simulink model "commander_old"  (R2024b)
(part 3 of 3)

    |     set_health_flags(SUBSYSTEM_TYPE_DIFFPRESSURE, present, ~optional_aspd, success, vehicle_status_out_);
    |     ret = success;
    |     return
    | end
    | 
    | %% Check if airspeed is declared valid or not by airspeed selector.
    | if ~isfinite(airspeed_validated.calibrated_airspeed_m_s) && report_fail
    |     sprintf("mavlink_log_critical, Preflight Fail: Airspeed invalid.");
    | end
    | present = true;
    | success = false;
    | set_health_flags(SUBSYSTEM_TYPE_DIFFPRESSURE, present, ~optional_aspd, success, vehicle_status_out_);
    | ret = success;
    | return
    | 
    | %% Check if airspeed is higher than maximally accepted while the vehicle is landed / not flying
    | %% Negative and positive offsets are considered. Do not check anymore while arming because pitot cover
    | %% might have been removed.
    | if max_aspd_check_en && fabsf(airspeed_validated.calibrated_airspeed_m_s) > arming_max_aspd_allowed && ...
    |         prearm && report_fail
    |     sprintf("mavlink_log_critical, Preflight Fail: check Airspeed Cal or pitot");
    | end
    | 
    | present = true;
    | success = false;
    | set_health_flags(SUBSYSTEM_TYPE_DIFFPRESSURE, present, ~optional_aspd, success, vehicle_status_out_);
    | ret = success;
    | return
    | 
    | end
  function ret = rcCheck(is_report_rc_fail, isVTOL):
    | function ret = rcCheck(is_report_rc_fail, isVTOL)
    | 
    | map_fail_count = 0;
    | total_fail_count = 0;
    | 
    | % if VTOL, check transition switch mapping
    | if isVTOL
    |     if RC_MAP_TRANS_SW == 0xffff && is_report_rc_fail
    |         sprintf("mavlink_log_critical, RC_MAP_TRANS_SW PARAMETER MISSING.");
    |         map_fail_count = map_fail_count + 1;
    |     elseif RC_MAP_TRANS_SW < 1
    |         if is_report_rc_fail
    |             sprintf("mavlink_log_critical, Transition switch RC_MAP_TRANS_SW not set.");
    |         end
    |         map_fail_count = map_fail_count + 1;
    |     end
    | 
    |     % first check channel mappings
    |     % 暂不实现
    | 
    |     channels_failed = 0;
    |     count = 0;
    | 
    |     % min values
    |     RC_INPUT_MIN_SETS = [RC1_MIN, RC2_MIN, RC3_MIN, RC4_MIN, RC5_MIN, RC6_MIN, ...
    |         RC7_MIN, RC8_MIN, RC9_MIN, RC10_MIN, RC11_MIN, RC12_MIN, ...
    |         RC13_MIN, RC14_MIN, RC15_MIN, RC16_MIN, RC17_MIN, RC18_MIN];
    | 
    |     % trim values
    |     RC_INPUT_TRIM_SETS = [RC1_TRIM, RC2_TRIM, RC3_TRIM, RC4_TRIM, RC5_TRIM, RC6_TRIM, ...
    |         RC7_TRIM, RC8_TRIM, RC9_TRIM, RC10_TRIM, RC11_TRIM, RC12_TRIM, ...
    |         RC13_TRIM, RC14_TRIM, RC15_TRIM, RC16_TRIM, RC17_TRIM, RC18_TRIM];
    | 
    |     % max values
    |     RC_INPUT_MAX_SETS = [RC1_MAX, RC2_MAX, RC3_MAX, RC4_MAX, RC5_MAX, RC6_MAX, ...
    |         RC7_MAX, RC8_MAX, RC9_MAX, RC10_MAX, RC11_MAX, RC12_MAX, ...
    |         RC13_MAX, RC14_MAX, RC15_MAX, RC16_MAX, RC17_MAX, RC18_MAX];
    | 
    |     % channel reverse
    |     RC_INPUT_REVERSE_SETS = [RC1_REV, RC2_REV, RC3_REV, RC4_REV, RC5_REV, RC6_REV, ...
    |         RC7_REV, RC8_REV, RC9_REV, RC10_REV, RC11_REV, RC12_REV, ...
    |         RC13_REV, RC14_REV, RC15_REV, RC16_REV, RC17_REV, RC18_REV];
    | 
    |     % channel deadzone
    |     RC_INPUT_DEADZONE_SETS = [RC1_DZ, RC2_DZ, RC3_DZ, RC4_DZ, RC5_DZ, RC6_DZ, ...
    |         RC7_DZ, RC8_DZ, RC9_DZ, RC10_DZ, RC11_DZ, RC12_DZ, ...
    |         RC13_DZ, RC14_DZ, RC15_DZ, RC16_DZ, RC17_DZ, RC18_DZ];
    | 
    |     for i = 1:uint8(PX4_INPUT_RC.RC_INPUT_MAX_CHANNELS)
    |         %% 检查MIN值的合理性
    |         if RC_INPUT_MIN_SETS(i) < RC_INPUT_LOWEST_MIN_US
    |             count = count + 1;
    |             if is_report_rc_fail
    |                 sprintf("mavlink_log_critical, RC_ERROR: RC%u_MIN < %d", i, RC_INPUT_LOWEST_MIN_US);
    |             end
    |         end
    | 
    |         %% 检查MAX值的合理性
    |         if RC_INPUT_MAX_SETS(i) > RC_INPUT_HIGHEST_MAX_US
    |             count = count + 1;
    |             if is_report_rc_fail
    |                 sprintf("mavlink_log_critical, RC_ERROR: RC%u_MAX < %d", i, RC_INPUT_HIGHEST_MAX_US);
    |             end
    |         end
    | 
    |         %% 检查TRIM与MIN数值的合理性
    |         if RC_INPUT_TRIM_SETS(i) < RC_INPUT_MIN_SETS(i)
    |             count = count + 1;
    |             if is_report_rc_fail
    |                 sprintf("mavlink_log_critical, RC ERROR: RC%d_TRIM < MIN (%d/%d).", int8(i), int16(RC_INPUT_TRIM_SETS(i)), int16(RC_INPUT_MIN_SETS(i)));
    |             end
    |         end
    | 
    |         %% 检查TRIM与MAX数值的合理性
    |         if RC_INPUT_TRIM_SETS(i) > RC_INPUT_MAX_SETS(i)
    |             count = count + 1;
    |             if is_report_rc_fail
    |                 sprintf("mavlink_log_critical, RC ERROR: RC%d_TRIM > MAX (%d/%d).", int8(i), int16(RC_INPUT_TRIM_SETS(i)), int16(RC_INPUT_MAX_SETS(i)));
    |             end
    |         end
    | 
    |         %% 检查死区的合理性
    |         if RC_INPUT_DEADZONE_SETS(i) > RC_INPUT_MAX_DEADZONE_US
    |             count = count + 1;
    |             if is_report_rc_fail
    |                 sprintf("mavlink_log_critical, RC ERROR: RC%d_DZ > %d.", int8(i), int16(RC_INPUT_MAX_DEADZONE_US));
    |             end
    |         end
    | 
    |         total_fail_count = total_fail_count + count;
    | 
    |     end
    | 
    | end
    | 
    | ret = total_fail_count;
    | 
    | end % function end
  function ret = powerCheck(report_power_fail, prearm):
    | function ret = powerCheck(report_power_fail, prearm)
    | 
    | ret = true;
    | 
    | if ~prearm
    |     % Ignore power check after arming.
    |     ret = true;
    |     return
    | end
    | 
    | if vehicle_status_out_.hil_state == PX4_VEHICLE_STATUS.HIL_STATE_ON
    |     % Ignore power check in HITL.
    |     ret = true;
    |     return
    | end
    | 
    | if system_power.timestamp ~= 0
    |     %% system_power主题有效
    |     required_power_module_count = 0;
    |     required_power_module_count = COM_POWER_COUNT;
    | 
    |     % Check avionics rail voltages (if USB isn't connected)
    |     if ~system_power.usb_connected
    | 
    |         avionics_power_rail_voltage = system_power.voltage5v_v;
    | 
    |         if avionics_power_rail_voltage < 4.5
    |             ret = false;
    |             if report_power_fail
    |                 sprintf("mavlink_log_critical, Preflight Fail: Avionics Power low: %6.2f Volt", single(avionics_power_rail_voltage));
    |             end
    |         elseif avionics_power_rail_voltage < 4.8 && report_power_fail
    |             sprintf("mavlink_log_critical, CAUTION: Avionics Power low: %6.2f Volt", single(avionics_power_rail_voltage));
    |         elseif avionics_power_rail_voltage > 5.4 && report_power_fail
    |             sprintf("mavlink_log_critical, CAUTION: Avionics Power high: %6.2f Volt", single(avionics_power_rail_voltage));
    |         end
    | 
    |         power_module_count = countSetBits(system_power.brick_valid);
    | 
    |         if power_module_count < required_power_module_count
    |             ret = false;
    |             if report_power_fail
    |                 sprintf("mavlink_log_critical, Power redundancy not met: %d instead of %d PRId32", int8(power_module_count), int8(required_power_module_count));
    |             end
    |         end
    | 
    |     elseif report_power_fail
    |         %% 主题无效
    |         sprintf("mavlink_log_critical, system power unavailable");
    |         ret = false;
    |         return
    | 
    |     end
    | 
    | end
    | 
    | end
    | 
    | %% 统计uint8的数据n中有多少位置1
    | function ret = countSetBits(n)
    | 
    | count = 0;
    | 
    | while n
    |     if bitand(uint8(n), uint8(1)) == 1
    |         count = count + 1;
    |     end
    |     n = bitshift(n, -1);
    | end
    | 
    | ret = count;
    | 
    | end
  function ret = failureDetectorCheck(report_failure_fail):
    | function ret = failureDetectorCheck(report_failure_fail)
    | 
    | ret = true;
    | 
    | % Ignore failure detector check after arming
    | if ~prearm_
    |     ret = true;
    |     return
    | end
    | 
    | if vehicle_status_out_.failure_detector_status ~= PX4_VEHICLE_STATUS.FAILURE_NONE
    | 
    |     if report_failure_fail
    |         if bitand(vehicle_status_out_.failure_detector_status, uint8(PX4_VEHICLE_STATUS.FAILURE_ROLL))
    |             sprintf("mavlink_log_critical, Preflight Fail: Roll failure detected");
    |         end
    | 
    |         if bitand(vehicle_status_out_.failure_detector_status, uint8(PX4_VEHICLE_STATUS.FAILURE_PITCH))
    |             sprintf("mavlink_log_critical, Preflight Fail: Pitch failure detected");
    |         end
    | 
    |         if bitand(vehicle_status_out_.failure_detector_status, uint8(PX4_VEHICLE_STATUS.FAILURE_ALT))
    |             sprintf("mavlink_log_critical, Preflight Fail: Altitude failure detected");
    |         end
    | 
    |         if bitand(vehicle_status_out_.failure_detector_status, uint8(PX4_VEHICLE_STATUS.FAILURE_EXT))
    |             sprintf("mavlink_log_critical, Preflight Fail: Parachute failure detected");
    |         end
    | 
    |         if bitand(vehicle_status_out_.failure_detector_status, uint8(PX4_VEHICLE_STATUS.FAILURE_ARM_ESC))
    |             sprintf("mavlink_log_critical, Preflight Fail: ESC failure detected");
    |         end
    |     end
    | 
    |     ret = false;
    |     return
    | 
    | end
    | 
    | ret = true;
    | return
    | 
    | end
  function ret = ekf2Check(report_ekf_fail):
    | function ret = ekf2Check(report_ekf_fail)
    | 
    | ret = true; % start with a pass and change to a fail if any test fails
    | 
    | mag_strength_check_enabled  = COM_ARM_MAG_STR;
    | hgt_test_ratio_limit        = COM_ARM_EKF_HGT;
    | vel_test_ratio_limit        = COM_ARM_EKF_VEL;
    | pos_test_ratio_limit        = COM_ARM_EKF_POS;
    | mag_test_ratio_limit        = COM_ARM_EKF_YAW;
    | arm_without_gps             = COM_ARM_WO_GPS;
    | 
    | gps_success = true;
    | gps_present = true;
    | 
    | % Get estimator status data if available and exit with a fail recorded if not
    | if vehicle_status_out_.timestamp == 0
    |     ret = false;
    |     set_health_flags(SUBSYSTEM_TYPE_GPS, gps_present, ~arm_without_gps, ret, vehicle_status_out_);
    |     return
    | end
    | 
    | % Check if preflight check performed by estimator has failed
    | if estimator_status.pre_flt_fail_innov_heading || estimator_status.pre_flt_fail_innov_vel_horiz || ...
    |         estimator_status.pre_flt_fail_innov_vel_vert || estimator_status.pre_flt_fail_innov_height
    | 
    |     if report_ekf_fail
    |         if estimator_status.pre_flt_fail_innov_heading
    |             sprintf("mavlink_log_critical, Preflight Fail: heading estimate not stable");
    |         elseif estimator_status.pre_flt_fail_innov_vel_horiz
    |             sprintf("mavlink_log_critical, Preflight Fail: horizontal velocity estimate not stable");
    |         elseif estimator_status.pre_flt_fail_innov_vel_vert
    |             sprintf("mavlink_log_critical, Preflight Fail: vertical velocity estimate not stable");
    |         elseif estimator_status.pre_flt_fail_innov_height
    |             sprintf("mavlink_log_critical, Preflight Fail: height estimate not stable");
    |         end
    |     end
    | 
    |     ret = false;
    |     set_health_flags(SUBSYSTEM_TYPE_GPS, gps_present, ~arm_without_gps, ret, vehicle_status_out_);
    |     return
    | 
    | end
    | 
    | %% 磁力计干扰检查
    | if mag_strength_check_enabled == 1 && estimator_status.pre_flt_fail_mag_field_disturbed
    |     if report_ekf_fail
    |         sprintf("mavlink_log_critical, Preflight Fail: strong magnetic interference detected");
    |     end
    |     ret = false;
    |     set_health_flags(SUBSYSTEM_TYPE_GPS, gps_present, ~arm_without_gps, ret, vehicle_status_out_);
    |     return
    | end
    | 
    | %% check vertical position innovation test ratio
    | if estimator_status.hgt_test_ratio > hgt_test_ratio_limit
    |     if report_ekf_fail
    |         sprintf("Preflight Fail: Height estimate error");
    |     end
    |     ret = false;
    |     set_health_flags(SUBSYSTEM_TYPE_GPS, gps_present, ~arm_without_gps, ret, vehicle_status_out_);
    |     return
    | end
    | 
    | %% check velocity innovation test ratio
    | if estimator_status.vel_test_ratio > vel_test_ratio_limit
    |     if report_ekf_fail
    |         sprintf("mavlink_log_critical, Preflight Fail: Velocity estimate error");
    |         ret = false;
    |         set_health_flags(SUBSYSTEM_TYPE_GPS, gps_present, ~arm_without_gps, ret, vehicle_status_out_);
    |         return
    |     end
    | end
    | 
    | %% check horizontal position innovation test ratio
    | if estimator_status.pos_test_ratio > pos_test_ratio_limit
    |     if report_ekf_fail
    |         sprintf("Preflight Fail: Position estimate error");
    |     end
    |     ret = false;
    |     set_health_flags(SUBSYSTEM_TYPE_GPS, gps_present, ~arm_without_gps, ret, vehicle_status_out_);
    |     return
    | end
    | 
    | %% check magnetometer innovation test ratio
    | if estimator_status.mag_test_ratio > mag_test_ratio_limit
    |     if report_ekf_fail
    |         sprintf("Preflight Fail: Yaw estimate error");
    |     end
    |     ret = false;
    |     set_health_flags(SUBSYSTEM_TYPE_GPS, gps_present, ~arm_without_gps, ret, vehicle_status_out_);
    |     return
    | end
    | 
    | %% If GPS aiding is required, declare fault condition if the required GPS quality checks are failing
    | ekf_gps_fusion = bitand(estimator_status.control_mode_flags, bitshift(1, PX4_ESTIMATOR_STATUS.CS_GPS));
    | ekf_gps_check_fail = estimator_status.gps_check_fail_flags > 0;
    | 
    | gps_success = ekf_gps_fusion; % default to success if gps data is fused
    | 
    | if ekf_gps_check_fail
    | 
    |     if report_ekf_fail
    |         % Only report the first failure to avoid spamming
    |         if bitand(estimator_status.gps_check_fail_flags, bitshift(1, PX4_ESTIMATOR_STATUS.GPS_CHECK_FAIL_GPS_FIX)) && ~arm_without_gps
    |             sprintf("mavlink_log_critical, Preflight Fail: GPS fix too low");
    |         elseif bitand(estimator_status.gps_check_fail_flags, bitshift(1, PX4_ESTIMATOR_STATUS.GPS_CHECK_FAIL_MIN_SAT_COUNT)) && ~arm_without_gps
    |             sprintf("mavlink_log_critical, Preflight Fail: not enough GPS Satellites");
    |         elseif bitand(estimator_status.gps_check_fail_flags, bitshift(1, PX4_ESTIMATOR_STATUS.GPS_CHECK_FAIL_MAX_PDOP)) && ~arm_without_gps
    |             sprintf("mavlink_log_critical, Preflight Fail: GPS PDOP too high");
    |         elseif bitand(estimator_status.gps_check_fail_flags, bitshift(1, PX4_ESTIMATOR_STATUS.GPS_CHECK_FAIL_MAX_HORZ_ERR)) && ~arm_without_gps
    |             sprintf("mavlink_log_critical, Preflight Fail: GPS Horizontal Pos Error too high");
    |         elseif bitand(estimator_status.gps_check_fail_flags, bitshift(1, PX4_ESTIMATOR_STATUS.GPS_CHECK_FAIL_MAX_VERT_ERR)) && ~arm_without_gps
    |             sprintf("mavlink_log_critical, Preflight Fail: GPS Vertical Pos Error too high");
    |         elseif bitand(estimator_status.gps_check_fail_flags, bitshift(1, PX4_ESTIMATOR_STATUS.GPS_CHECK_FAIL_MAX_SPD_ERR)) && ~arm_without_gps
    |             sprintf("mavlink_log_critical, Preflight Fail: GPS Speed Accuracy too low");
    |         elseif bitand(estimator_status.gps_check_fail_flags, bitshift(1, PX4_ESTIMATOR_STATUS.GPS_CHECK_FAIL_MAX_HORZ_DRIFT)) && ~arm_without_gps
    |             sprintf("mavlink_log_critical, Preflight Fail: GPS Horizontal Pos Drift too high");
    |         elseif bitand(estimator_status.gps_check_fail_flags, bitshift(1, PX4_ESTIMATOR_STATUS.GPS_CHECK_FAIL_MAX_VERT_DRIFT)) && ~arm_without_gps
    |             sprintf("mavlink_log_critical, Preflight Fail: GPS Vertical Pos Drift too high");
    |         elseif bitand(estimator_status.gps_check_fail_flags, bitshift(1, PX4_ESTIMATOR_STATUS.GPS_CHECK_FAIL_MAX_HORZ_SPD_ERR)) && ~arm_without_gps
    |             sprintf("mavlink_log_critical, Preflight Fail: GPS Hor Speed Drift too high");
    |         elseif bitand(estimator_status.gps_check_fail_flags, bitshift(1, PX4_ESTIMATOR_STATUS.GPS_CHECK_FAIL_MAX_VERT_SPD_ERR)) && ~arm_without_gps
    |             sprintf("mavlink_log_critical, Preflight Fail: GPS Vert Speed Drift too high");
    |         else
    |             if ~ekf_gps_fusion
    |                 % Likely cause unknown
    |                 sprintf("mavlink_log_critical, Preflight Fail: Estimator not using GPS");
    |                 gps_present = false;
    |             else
    |                 % if we land here there was a new flag added and the code not updated. Show a generic message.
    |                 sprintf("mavlink_log_critical, Preflight Fail: Poor GPS Quality");
    |             end
    |         end
    | 
    |         gps_success = false;
    | 
    |         if ~arm_without_gps
    |             ret = false;
    |             set_health_flags(SUBSYSTEM_TYPE_GPS, gps_present, ~arm_without_gps, gps_success, vehicle_status_out_);
    |             return
    |         end
    |     end
    | 
    | end
    | 
    | end % function end
  function ret = ekf2CheckSensorBias(report_bias_fail):
    | function ret = ekf2CheckSensorBias(report_bias_fail)
    | 
    | % Get estimator states data if available and exit with a fail recorded if not
    | % uORB::SubscriptionData<estimator_selector_status_s> estimator_selector_status_sub{ORB_ID(estimator_selector_status)};
    | % uORB::SubscriptionData<estimator_sensor_bias_s> estimator_sensor_bias_sub{ORB_ID(estimator_sensor_bias), estimator_selector_status_sub.get().primary_instanceend};
    | 
    | if (getSimulationTime*1e+6 - estimator_sensor_bias.timestamp) < 30*1e+6
    | 
    |     %% check accelerometer bias estimates
    |     if estimator_sensor_bias.accel_bias_valid
    |         ekf_ab_test_limit = 0.75 * estimator_sensor_bias.accel_bias_limit;
    |         for axis_index = 1:3
    |             % allow for higher uncertainty in estimates for axes that are less observable to prevent false positives
    |             % adjust test threshold by 3-sigma
    |             test_uncertainty = 3.0 * sqrt(max(estimator_sensor_bias.accel_bias_variance(axis_index), 0.0));
    |             if abs(estimator_sensor_bias.accel_bias(axis_index)) > (ekf_ab_test_limit + test_uncertainty)
    |                 if report_bias_fail
    |                     sprintf("PX4_ERR, accel bias (axis %d): |%f| > %f + %f", int8(axis_index), ...
    |                         single(estimator_sensor_bias.accel_bias(axis_index)), single(ekf_ab_test_limit), single(test_uncertainty));
    |                     sprintf("mavlink_log_critical, Preflight Fail: High Accelerometer Bias");
    |                 end
    |                 ret = false;
    |                 return
    |             end
    |         end
    |     end
    | 
    |     %% check gyro bias estimates
    |     if estimator_sensor_bias.gyro_bias_valid
    |         ekf_gb_test_limit = 0.75 * estimator_sensor_bias.gyro_bias_limit;
    |         for axis_index = 1:3
    |             % allow for higher uncertainty in estimates for axes that are less observable to prevent false positives
    |             % adjust test threshold by 3-sigma
    |             test_uncertainty = 3.0 * sqrt(max(estimator_sensor_bias.gyro_bias_variance(axis_index), 0.0));
    |             if abs(estimator_sensor_bias.gyro_bias(axis_index)) > (ekf_gb_test_limit + test_uncertainty)
    |                 if report_bias_fail
    |                     sprintf("PX4_ERR, gyro bias (axis %d): |%f| > %f + %f", int8(axis_index), ...
    |                         single(estimator_sensor_bias.gyro_bias(axis_index)), single(ekf_gb_test_limit), single(test_uncertainty));
    |                     sprintf("mavlink_log_critical, Preflight Fail: High Gyro Bias");
    |                 end
    |                 ret = false;
    |                 return
    |             end
    |         end
    |     end
    | 
    | end
    | 
    | ret = true;
    | 
    | end % function end
  function ret = manualCheck(report_manual_fail):
    | function ret = manualCheck(report_manual_fail)
    | 
    | ret = true;
    | 
    | if manual_control_switches.timestamp ~= 0
    | 
    |     % check action switches
    |     if manual_control_switches.return_switch == PX4_MANUAL_CONTROL_SWITCHES.SWITCH_POS_ON
    |         ret = false;
    |         if report_manual_fail
    |             sprintf("mavlink_log_critical, Failure: RTL switch engaged");
    |         end
    |     end
    | 
    |     if manual_control_switches.kill_switch == PX4_MANUAL_CONTROL_SWITCHES.SWITCH_POS_ON
    |         ret = false;
    |         if report_manual_fail
    |             sprintf("mavlink_log_critical, Failure: Kill switch engaged");
    |         end
    |     end
    | 
    |     if manual_control_switches.gear_switch == PX4_MANUAL_CONTROL_SWITCHES.SWITCH_POS_ON
    |         ret = false;
    |         if (report_manual_fail)
    |             sprintf("mavlink_log_critical, Failure: Landing gear switch set in UP position");
    |         end
    |     end
    |     
    | end
    | 
    | end
  function ret = cpuCheck(report_cpu_fail):
    | function ret = cpuCheck(report_cpu_fail)
    | 
    | ret = true;
    | 
    | cpuload_percent_max = COM_CPU_MAX;
    | 
    | if cpuload_percent_max > 0.0
    | 
    |     if (getSimulationTime*1e+6 - cpuload.timestamp) > 2*1e+6
    |         ret = false;
    |         if report_cpu_fail
    |             sprintf("mavlink_log_critical, Fail: No CPU load information");
    |         end
    |     end
    | 
    |     cpuload_percent = cpuload.load * 100;
    | 
    |     if cpuload_percent > cpuload_percent_max
    |         ret = false;
    |         if report_cpu_fail
    |             sprintf("mavlink_log_critical, Fail: CPU load too high: %f", single(cpuload_percent));
    |         end
    |     end
    | 
    | end
    | 
    | end
  function ret = is_fixed_wing(current_status):
    | function ret = is_fixed_wing(current_status)
    | 
    | ret = current_status.system_type == VEHICLE_TYPE_FIXED_WING;
    | 
    | end
  function ret = is_multirotor(current_status):
    | function ret = is_multirotor(current_status)
    | 
    | ret = ((current_status.system_type == VEHICLE_TYPE_QUADROTOR) || ...
    |     (current_status.system_type == VEHICLE_TYPE_HEXAROTOR) || ...
    |     (current_status.system_type == VEHICLE_TYPE_OCTOROTOR) || ...
    |     (current_status.system_type == VEHICLE_TYPE_TRICOPTER));
    | 
    | end
  function ret = is_ground_rover(current_status):
    | function ret = is_ground_rover(current_status)
    | 
    | ret = current_status.system_type == VEHICLE_TYPE_GROUND_ROVER;
    | 
    | end
  function get_circuit_breaker_params:
    | function get_circuit_breaker_params()
    | 
    | vehicle_status_flags_out_.circuit_breaker_engaged_power_check = (CBRK_SUPPLY_CHK == CBRK_SUPPLY_CHK_KEY);
    | vehicle_status_flags_out_.circuit_breaker_engaged_usb_check = (CBRK_USB_CHK == CBRK_USB_CHK_KEY);
    | vehicle_status_flags_out_.circuit_breaker_engaged_airspd_check = (CBRK_AIRSPD_CHK == CBRK_AIRSPD_CHK_KEY);
    | vehicle_status_flags_out_.circuit_breaker_engaged_enginefailure_check = (CBRK_ENGINEFAIL == CBRK_ENGINEFAIL_KEY);
    | vehicle_status_flags_out_.circuit_breaker_flight_termination_disabled = (CBRK_FLIGHTTERM == CBRK_FLIGHTTERM_KEY);
    | vehicle_status_flags_out_.circuit_breaker_engaged_posfailure_check = (CBRK_VELPOSERR == CBRK_VELPOSERR_KEY);
    | vehicle_status_flags_out_.circuit_breaker_vtol_fw_arming_check = (CBRK_VTOLARMING == CBRK_VTOLARMING_KEY);
    | 
    | end
  function update_vtol_status:
    | function update_vtol_status()
    | 
    | % vtol status changed
    | vehicle_status_out_.vtol_fw_permanent_stab = vtol_status.fw_permanent_stab;
    | 
    | % Make sure that this is only adjusted if vehicle really is of type vtol
    | if is_vtol(vehicle_status_out_)
    | 
    |     % Check if there has been any change while updating the flags
    |     if vtol_status.vtol_in_rw_mode % 转换和多旋翼阶段
    |         new_vehicle_type = uint8(PX4_VEHICLE_STATUS.VEHICLE_TYPE_ROTARY_WING);
    |     else  % 纯固定翼
    |         new_vehicle_type = uint8(PX4_VEHICLE_STATUS.VEHICLE_TYPE_FIXED_WING);
    |     end
    | 
    |     if new_vehicle_type ~= vehicle_status_out_.vehicle_type
    |         vehicle_status_out_.vehicle_type = new_vehicle_type;
    |         g_status_changed = true;
    |     end
    | 
    |     if vehicle_status_out_.in_transition_mode ~= vtol_status.vtol_in_trans_mode
    |         vehicle_status_out_.in_transition_mode = vtol_status.vtol_in_trans_mode;
    |         g_status_changed = true;
    |     end
    | 
    |     if vehicle_status_out_.in_transition_to_fw ~= vtol_status.in_transition_to_fw
    |         vehicle_status_out_.in_transition_to_fw = vtol_status.in_transition_to_fw;
    |         g_status_changed = true;
    |     end
    | 
    |     if vehicle_status_flags_out_.vtol_transition_failure ~= vtol_status.vtol_transition_failsafe
    |         vehicle_status_flags_out_.vtol_transition_failure = vtol_status.vtol_transition_failsafe;
    |         g_status_changed = true;
    |     end
    | 
    |     should_soft_stop = (vehicle_status_out_.vehicle_type ~= uint8(PX4_VEHICLE_STATUS.VEHICLE_TYPE_ROTARY_WING));
    | 
    |     if actuator_armed_out_.soft_stop ~= should_soft_stop
    |         actuator_armed_out_.soft_stop = should_soft_stop;
    |         g_status_changed = true;
    |     end
    | 
    | end
    | 
    | end % function end
  function last_esc_updated = esc_status_check:
    | function last_esc_updated = esc_status_check
    | 
    | persistent last_esc_online_flags
    | persistent last_esc_failure
    | 
    | if isempty(last_esc_online_flags)
    |     last_esc_online_flags = uint8(0);
    | end
    | 
    | if isempty(last_esc_failure)
    |     last_esc_failure = uint8(zeros(1, uint8(PX4_ESC_STATUS.CONNECTED_ESC_MAX)));
    | end
    | 
    | last_esc_updated = esc_status.timestamp;
    | 
    | if esc_status.esc_count > 0
    | 
    |     online_bitmask = bitshift(1, esc_status.esc_count) - 1;
    | 
    |     %% Check if ALL the ESCs are online
    |     if online_bitmask == esc_status.esc_online_flags
    |         vehicle_status_flags_out_.condition_escs_error = false;
    |         last_esc_online_flags = esc_status.esc_online_flags;
    |     elseif esc_status.esc_online_flags == last_esc_online_flags
    |         % Avoid checking the status if the flags are the same or if the mixer has not yet been loaded in the ESC driver
    |         vehicle_status_flags_out_.condition_escs_error = true;
    |     elseif esc_status.esc_online_flags < last_esc_online_flags
    |         % Only warn the user when an ESC goes from ONLINE to OFFLINE. This is done to prevent showing Offline ESCs warnings at boot
    |         for index = 1:esc_status.esc_count
    |             if bitand(esc_status.esc_online_flags, bitshift(1,index-1)) == 0
    |                 sprintf("mavlink_log_critical, %d offline", int8(index));
    |             end
    |         end
    |         last_esc_online_flags = esc_status.esc_online_flags;
    |         vehicle_status_flags_out_.condition_escs_error = true;
    |     end
    | 
    |     vehicle_status_flags_out_.condition_escs_failure = false;
    | 
    |     for index = 1:esc_status.esc_count
    | 
    |         if esc_status.esc(index).failures > PX4_ESC_REPORT.FAILURE_NONE
    |             vehicle_status_flags_out_.condition_escs_failure = true;
    | 
    |             if esc_status.esc(index).failures ~= last_esc_failure(index)
    | 
    |                 if bitand(esc_status.esc(index).failures, uint8(PX4_ESC_REPORT.FAILURE_OVER_CURRENT_MASK))
    |                     sprintf("mavlink_log_critical ESC%d: over current", int8(index));
    |                 end
    | 
    |                 if bitand(esc_status.esc(index).failures, uint8(PX4_ESC_REPORT.FAILURE_OVER_VOLTAGE_MASK))
    |                     sprintf("mavlink_log_critical ESC%d: over voltage", int8(index));
    |                 end
    | 
    |                 if bitand(esc_status.esc(index).failures, uint8(PX4_ESC_REPORT.FAILURE_OVER_TEMPERATURE_MASK))
    |                     sprintf("mavlink_log_critical ESC%d: over temperature", int8(index));
    |                 end
    | 
    |                 if bitand(esc_status.esc(index).failures, uint8(PX4_ESC_REPORT.FAILURE_OVER_RPM_MASK))
    |                     sprintf("mavlink_log_critical ESC%d: over RPM", int8(index));
    |                 end
    | 
    |                 if bitand(esc_status.esc(index).failures, uint8(PX4_ESC_REPORT.FAILURE_INCONSISTENT_CMD_MASK))
    |                     sprintf("mavlink_log_critical ESC%d: command inconsistency", int8(index));
    |                 end
    | 
    |                 if bitand(esc_status.esc(index).failures, uint8(PX4_ESC_REPORT.FAILURE_MOTOR_STUCK_MASK))
    |                     sprintf("mavlink_log_critical ESC%d: motor stuck", int8(index));
    |                 end
    | 
    |                 if bitand(esc_status.esc(index).failures, uint8(PX4_ESC_REPORT.FAILURE_GENERIC_MASK))
    |                     sprintf("mavlink_log_critical ESC%d: generic failure - code %d", int8(index), int16(esc_status.esc(index).esc_state));
    |                 end
    | 
    |             end
    | 
    |             last_esc_failure(index) = esc_status.esc(index).failures;
    |         end
    | 
    |     end
    | 
    | end
    | 
    | end % function end
  function ekf_status_check:
    | function ekf_status_check()
    | 
    | % persistent parameters
    | persistent heading_reset_counter
    | persistent time_last_innov_fail
    | persistent time_last_innov_pass
    | 
    | if isempty(heading_reset_counter)
    |     heading_reset_counter = uint8(0);
    | end
    | 
    | if isempty(time_last_innov_fail)
    |     time_last_innov_fail = uint64(0);
    | end
    | 
    | if isempty(time_last_innov_pass)
    |     time_last_innov_pass = uint64(0);
    | end
    | 
    | % Check if quality checking of position accuracy and consistency is to be performed
    | % circuit_breaker_engaged_posfailure_check: set to true when the position valid checks have been disabled
    | run_quality_checks = ~vehicle_status_flags_out_.circuit_breaker_engaged_posfailure_check;
    | if local_position.heading_reset_counter ~= heading_reset_counter
    |     if vehicle_status_flags_out_.condition_home_position_valid
    |         updateHomePositionYaw(home_position.yaw + local_position.delta_heading);
    |     end
    |     heading_reset_counter = local_position.heading_reset_counter;
    | end
    | 
    | mag_fault_prev = bitand(estimator_status.control_mode_flags, bitshift(1, PX4_ESTIMATOR_STATUS.CS_MAG_FAULT));
    | 
    | %% use primary estimator_status, but we use only one ekf
    | if hasChanged(estimator_status.timestamp)
    | 
    |     % Check for a magnetomer fault and notify the user
    |     mag_fault = bitand(estimator_status.control_mode_flags, bitshift(1, PX4_ESTIMATOR_STATUS.CS_MAG_FAULT));
    |     if ~mag_fault_prev && mag_fault
    |         sprintf("mavlink_log_critical, Stopping compass use~ Check calibration on landing");
    |         set_health_flags(SUBSYSTEM_TYPE_MAG, true, true, false, vehicle_status_out_);
    |     end
    | 
    |     % Check estimator status for signs of bad yaw induced post takeoff navigation failure
    |     % for a short time interval after takeoff.
    |     % Most of the time, the drone can recover from a bad initial yaw using GPS-inertial
    |     % heading estimation (yaw emergency estimator) or GPS heading (fixed wings only), but
    |     % if this does not fix the issue we need to stop using a position controlled
    |     % mode to prevent flyaway crashes.
    |     if run_quality_checks && (vehicle_status_out_.vehicle_type == PX4_VEHICLE_STATUS.VEHICLE_TYPE_ROTARY_WING)
    | 
    |         if vehicle_status_out_.arming_state == PX4_VEHICLE_STATUS.ARMING_STATE_STANDBY
    |             nav_test_failed_ = false;
    |             nav_test_passed_ = false;
    |         else
    |             if ~nav_test_passed_
    |                 % Both test ratios need to pass/fail together to change the nav test status
    |                 innovation_pass = (estimator_status.vel_test_ratio < 1.0) && (estimator_status.pos_test_ratio < 1.0) && ...
    |                     (estimator_status.vel_test_ratio > eps) && (estimator_status.pos_test_ratio > eps);
    |                 innovation_fail = (estimator_status.vel_test_ratio >= 1.0) && (estimator_status.pos_test_ratio >= 1.0);
    | 
    |                 if innovation_pass
    |                     %% innovation_pass
    |                     time_last_innov_pass = uint64(getSimulationTime*1e+6);
    |                     % if nav status is unconfirmed, confirm yaw angle as passed after 30 seconds or achieving 5 m/s of speed
    |                     sufficient_time = (vehicle_status_out_.takeoff_time ~= 0) && ...
    |                         (uint64(getSimulationTime*1e+6 - vehicle_status_out_.takeoff_time) > 30*1e+6);
    |                     sufficient_speed = norm([local_position.vx, local_position.vy]) > 5.0;
    |                     % Even if the test already failed, allow it to pass if it did not fail during the last 10 seconds
    |                     if (uint64(getSimulationTime*1e+6 - time_last_innov_fail) > 10*1e+6) && ...
    |                             (sufficient_time || sufficient_speed)
    |                         nav_test_passed_ = true;
    |                         nav_test_failed_ = false;
    |                     end
    | 
    |                 elseif innovation_fail
    |                     %% innovation_fail
    |                     time_last_innov_fail = uint64(getSimulationTime*1e+6);
    |                     if (~nav_test_failed_ && uint64(getSimulationTime*1e+6) - time_last_innov_pass) > 2*1e+6
    |                         % if the innovation test has failed continuously, declare the nav as failed
    |                         nav_test_failed_ = true;
    |                         sprintf("mavlink_log_emergency, Navigation failure~ Land and recalibrate sensors");
    |                     end
    |                 end
    |             end
    |         end
    |     end
    | 
    | end
    | 
    | %% run position and velocity accuracy checks
    | % Check if quality checking of position accuracy and consistency is to be performed
    | if run_quality_checks
    |     UpdateEstimateValidity();
    | end
    | vehicle_status_flags_out_.condition_local_altitude_valid = local_position.z_valid && ...
    |     (uint64(getSimulationTime*1e+6) - local_position.timestamp) < (COM_POS_FS_DELAY*1e+6);
    | 
    | %% attitude
    | q = vehicle_attitude.q;
    | q_norm = q/norm(q);
    | vehicle_status_flags_out_.condition_attitude_valid = (uint64(getSimulationTime*1e+6) - vehicle_attitude.timestamp) < 1e+6 && ...
    |     norm(q-q_norm) < eps;
    | 
    | %% angular velocity
    | vehicle_status_flags_out_.condition_angular_velocity_valid = ...
    |     (uint64(getSimulationTime*1e+6) - angular_velocity.timestamp) < 1e+6 && ...
    |     isfinite(angular_velocity.xyz(1)) && ...
    |     isfinite(angular_velocity.xyz(2)) && ...
    |     isfinite(angular_velocity.xyz(3));
    | 
    | end % function end
    | 
    | %% updateHomePositionYaw
    | function updateHomePositionYaw(yaw)
    | 
    | home_position_out_.yaw = yaw;
    | home_position_out_.timestamp = uint64(getSimulationTime*1e+6);
    | 
    | end
    | 
    | %% UpdateEstimateValidity
    | function UpdateEstimateValidity()
    | 
    | % COM_POS_FS_EPH: This is the horizontal position error (EPH) threshold that will trigger a failsafe.
    | % The default is appropriate for a multicopter. Can be increased for a fixed-wing.
    | % Default: 5m
    | lpos_eph_threshold_adj = COM_POS_FS_EPH;
    | 
    | % relax local position eph threshold in operator controlled position mode
    | if (internal_state_out_.main_state == PX4_COMMANDER_STATE.MAIN_STATE_POSCTL) && ...
    |         ((vehicle_status_out_.nav_state == PX4_VEHICLE_STATUS.NAVIGATION_STATE_ALTCTL) || ...
    |         (vehicle_status_out_.nav_state == PX4_VEHICLE_STATUS.NAVIGATION_STATE_POSCTL))
    | 
    |     % Set the allowable position uncertainty based on combination of flight and estimator state
    |     % When we are in a operator demanded position control mode and are solely reliant on optical flow,
    |     % do not check position error because it will gradually increase throughout flight and the operator will compensate for the drift
    |     reliant_on_opt_flow = (bitand(estimator_status.control_mode_flags, bitshift(1, PX4_ESTIMATOR_STATUS.CS_OPT_FLOW)) && ...
    |         ~bitand(estimator_status.control_mode_flags, bitshift(1, PX4_ESTIMATOR_STATUS.CS_GPS)) && ...
    |         ~bitand(estimator_status.control_mode_flags, bitshift(1, PX4_ESTIMATOR_STATUS.CS_EV_POS)));
    | 
    |     if reliant_on_opt_flow
    |         lpos_eph_threshold_adj = single(inf);
    |     end
    | end
    | 
    | vehicle_status_flags_out_.condition_global_position_valid = ...
    |     check_posvel_validity(local_position.xy_valid && ~nav_test_failed_, ...
    |     global_position.eph, COM_POS_FS_EPH, ...
    |     global_position.timestamp, ...
    |     last_gpos_fail_time_us_, gpos_probation_time_us_, ...
    |     vehicle_status_flags_out_.condition_global_position_valid);
    | 
    | vehicle_status_flags_out_.condition_local_position_valid = ...
    |     check_posvel_validity(local_position.xy_valid && ~nav_test_failed_, ...
    |     local_position.eph, lpos_eph_threshold_adj, local_position.timestamp, ...
    |     last_lpos_fail_time_us_, lpos_probation_time_us_, ...
    |     vehicle_status_flags_out_.condition_local_position_valid);
    | 
    | vehicle_status_flags_out_.condition_local_velocity_valid = ...
    |     check_posvel_validity(local_position.v_xy_valid && ~nav_test_failed_, ...
    |     local_position.evh, COM_VEL_FS_EVH, local_position.timestamp, ...
    |     last_lvel_fail_time_us_, lvel_probation_time_us_, ...
    |     vehicle_status_flags_out_.condition_local_velocity_valid);
    | 
    | end
  function [batt_warn, batt_warn_inc_while_armed] = battery_check:
    | function [batt_warn, batt_warn_inc_while_armed] = battery_check()
    | 
    | batt_warn = uint8(0);
    | batt_warn_inc_while_armed = false;
    | 
    | if hasChanged(battery_status.timestamp)
    |     
    |     % 此处假定有1块电池connected
    |     num_connected_batteries = 1;
    |     
    |     % 假定所有的电池全为一样的，batteries此处设置为1块电池
    |     for i = 1:num_connected_batteries
    |         batteries(i) = battery_status;
    |     end
    |     
    |     worst_warning = uint8(PX4_BATTERY_STATUS.BATTERY_WARNING_NONE);
    |     oldest_update = uint64(getSimulationTime * 1e+6);
    |     
    |     battery_current_ = single(0.0);
    |     battery_level = single(0.0);
    |     
    |     % Only iterate over connected batteries. We don't care if a disconnected battery is not regularly publishing.
    |     for i = 1:num_connected_batteries
    |         if (batteries(i).warning > worst_warning)
    |             worst_warning = batteries(i).warning;
    |         end
    |         
    |         current_time_us = uint64(getSimulationTime * 1e+6);
    |         if (current_time_us - batteries(i).timestamp) > (current_time_us - oldest_update)
    |             oldest_update = batteries(i).timestamp;
    |         end
    |         
    |         % Sum up current from all batteries.
    |         battery_current_ = battery_current_ + batteries(i).current_filtered_a;
    |         
    |         % average levels from all batteries
    |         battery_level = battery_level + batteries(i).remaining;
    |     end
    |     
    |     battery_level = battery_level / num_connected_batteries;
    |     battery_usage_to_home = single(0.0);
    |     
    |     if uint64(getSimulationTime*1e+6) - rtl_flight_time.timestamp < 2*1e+6
    |         battery_usage_to_home = rtl_flight_time.rtl_limit_fraction;
    |     end
    |     
    |     battery_range_warning = uint8(PX4_BATTERY_STATUS.BATTERY_WARNING_NONE);
    | 
    |     if isfinite(battery_usage_to_home)
    |         
    |         battery_at_home = battery_level - battery_usage_to_home;
    |         if battery_at_home < BAT_CRIT_THR
    |             battery_range_warning = uint8(PX4_BATTERY_STATUS.BATTERY_WARNING_CRITICAL);
    |         elseif battery_at_home < BAT_LOW_THR
    |             battery_range_warning = uint8(PX4_BATTERY_STATUS.BATTERY_WARNING_LOW);
    |         end
    |         
    |         if battery_range_warning > worst_warning
    |             worst_warning = battery_range_warning;
    |         end
    |         
    |         batt_warn_inc_while_armed = false;
    |         update_internal_battery_state = false;
    |         
    |         if actuator_armed.armed
    |             if worst_warning > batt_warn
    |                 batt_warn_inc_while_armed = true;
    |                 update_internal_battery_state = true;
    |             elseif battery_warning ~= worst_warning
    |                 update_internal_battery_state = true;
    |             end
    |         end
    |         
    |         if update_internal_battery_state
    |             batt_warn = worst_warning;
    |         end
    |         
    |         % All connected batteries are regularly being published
    |         % There is at least one connected battery (in any slot)
    |         % No currently-connected batteries have any warning
    |         vehicle_status_flags_out_.condition_battery_healthy = (uint64(getSimulationTime * 1e+6) - oldest_update < 5 * 1e+6) && ...
    |             (num_connected_batteries > 0) && (batt_warn == uint8(PX4_BATTERY_STATUS.BATTERY_WARNING_NONE));
    |     end
    |     
    | end  % function end
  function battery_warning_critical:
    | function battery_warning_critical()
    | 
    | % switch low battery action
    | switch COM_LOW_BAT_ACT
    |     
    |     case BATTERY_FAILSAFE_WARNING
    |         sprintf("mavlink_log_critical, Critical battery level! landing advised");
    |         
    |     case BATTERY_FAILSAFE_RETURN || BATTERY_FAILSAFE_RETURN_OR_LAND
    |         if (status_flags.condition_global_position_valid && status_flags.condition_home_position_valid)
    |             if (~(internal_state_out_.main_state == uint8(PX4_COMMANDER_STATE.MAIN_STATE_AUTO_RTL) || ...
    |                     internal_state_out_.main_state == uint8(PX4_COMMANDER_STATE.MAIN_STATE_AUTO_LAND) || ...
    |                     internal_state_out_.main_state == uint8(PX4_COMMANDER_STATE.MAIN_STATE_AUTO_PRECLAND)))
    |                 internal_state_out_.main_state = uint8(PX4_COMMANDER_STATE.MAIN_STATE_AUTO_RTL);
    |                 internal_state_out_.timestamp = uint64(getSimulationTime * 1e+6);
    |                 sprintf("mavlink_log_critical, Critical battery level! executing RTL");
    |             end
    |         else
    |             if (~(internal_state_out_.main_state == uint8(PX4_COMMANDER_STATE.MAIN_STATE_AUTO_LAND) || ...
    |                     internal_state_out_.main_state == uint8(PX4_COMMANDER_STATE.MAIN_STATE_AUTO_PRECLAND)))
    |                 internal_state_out_.main_state = uint8(PX4_COMMANDER_STATE.MAIN_STATE_AUTO_LAND);
    |                 internal_state_out_.timestamp = uint64(getSimulationTime * 1e+6);
    |                 sprintf("mavlink_log_emergency, Critical battery level! can't execute RTL, landing instead");
    |             end
    |         end
    |         
    |     case BATTERY_FAILSAFE_LAND
    |         if (~(internal_state_out_.main_state == uint8(PX4_COMMANDER_STATE.MAIN_STATE_AUTO_LAND) || ...
    |                 internal_state_out_.main_state == uint8(PX4_COMMANDER_STATE.MAIN_STATE_AUTO_PRECLAND)))
    |             internal_state_out_.main_state = uint8(PX4_COMMANDER_STATE.MAIN_STATE_AUTO_LAND);
    |             internal_state_out_.timestamp = uint64(getSimulationTime * 1e+6);
    |             sprintf("mavlink_log_emergency, Critical battery level! landing");
    |         end
    |         
    | end
    | 
    | end % function end
  function battery_warning_emergency:
    | function battery_warning_emergency()
    | 
    | switch (COM_LOW_BAT_ACT)
    |     
    |     case BATTERY_FAILSAFE_WARNING
    |         sprintf("mavlink_log_emergency, Dangerous battery level! please land!");
    |         
    |     case BATTERY_FAILSAFE_RETURN
    |         if (vehicle_status_flags_out_.condition_global_position_valid && status_flags.condition_home_position_valid)
    |             if (~(internal_state_out_.main_state == uint8(PX4_COMMANDER_STATE.MAIN_STATE_AUTO_RTL) || ...
    |                     internal_state_out_.main_state == uint8(PX4_COMMANDER_STATE.MAIN_STATE_AUTO_LAND) || ...
    |                     internal_state_out_.main_state == uint8(PX4_COMMANDER_STATE.MAIN_STATE_AUTO_PRECLAND)))
    |                 internal_state_out_.main_state = uint8(PX4_COMMANDER_STATE.MAIN_STATE_AUTO_RTL);
    |                 internal_state_out_.timestamp = uint64(getSimulationTime * 1e+6);
    |                 sprintf("mavlink_log_critical, Dangerous battery level! executing RTL");
    |             elseif (~(internal_state_out_.main_state == uint8(PX4_COMMANDER_STATE.MAIN_STATE_AUTO_LAND) || ...
    |                     internal_state_out_.main_state == uint8(PX4_COMMANDER_STATE.MAIN_STATE_AUTO_PRECLAND)))
    |                 internal_state_out_.main_state = uint8(PX4_COMMANDER_STATE.MAIN_STATE_AUTO_LAND);
    |                 internal_state_out_.timestamp = uint64(getSimulationTime * 1e+6);
    |                 sprintf("mavlink_log_emergency, Dangerous battery level! can't execute RTL, landing instead");
    |             end
    |         end
    |         
    |     case {BATTERY_FAILSAFE_RETURN_OR_LAND, BATTERY_FAILSAFE_LAND}
    |         if (~(internal_state_out_.main_state == uint8(PX4_COMMANDER_STATE.MAIN_STATE_AUTO_LAND) || ...
    |                 internal_state_out_.main_state == uint8(PX4_COMMANDER_STATE.MAIN_STATE_AUTO_PRECLAND)))
    |             internal_state_out_.main_state = uint8(PX4_COMMANDER_STATE.MAIN_STATE_AUTO_LAND);
    |             internal_state_out_.timestamp = uint64(getSimulationTime * 1e+6);
    |             sprintf("mavlink_log_emergency, Dangerous battery level! landing");
    |         end
    | end
    | 
    | end % function end
  function evaluate_mission_state:
    | function evaluate_mission_state()
    | 
    | mission_instance_count = mission_result.instance_count;
    | 
    | % if mission_result is valid for the current mission
    | mission_result_ok = (mission_result.timestamp > boot_timestamp_) && (mission_result.instance_count > 0);
    | vehicle_status_flags_out_.condition_auto_mission_available = mission_result_ok && mission_result.valid;
    | 
    | if mission_result_ok
    |     
    |     %% check mission failure
    |     if vehicle_status_out_.mission_failure ~= mission_result.failure
    |         
    |         vehicle_status_out_.mission_failure = mission_result.failure;
    |         g_status_changed = true;
    |         
    |         if vehicle_status_out_.mission_failure
    |             sprintf("mavlink_log_critical, Mission cannot be completed")
    |         end
    |         
    |     end
    |     
    |     %% Only evaluate mission state if home is set
    |     if vehicle_status_flags_out_.condition_home_position_valid && hasChanged(mission_result.instance_count)
    |         
    |         if ~vehicle_status_flags_out_.condition_auto_mission_available
    |             % the mission is invalid
    |             tune_mission_fail(true);
    |         elseif mission_result.warning
    |             % the mission has a warning
    |             tune_mission_warn(true);
    |         else
    |             % the mission is valid
    |             tune_mission_ok(true);
    |         end
    |         
    |     end
    |     
    | end
    | 
    | end % function end
  function tune_mission_fail(use_buzzer):
    | function tune_mission_fail(use_buzzer)
    | 
    | % blink_msg_end = hrt_absolute_time() + BLINK_MSG_TIME;
    | % rgbled_set_color_and_mode(led_control_s::COLOR_RED, led_control_s::MODE_BLINK_FAST);
    | % 
    | if use_buzzer
    | %     set_tune(tune_control_s::TUNE_ID_NOTIFY_NEGATIVE);
    | end
    | 
    | end % function end
  function tune_mission_warn(use_buzzer):
    | function tune_mission_warn(use_buzzer)
    | 
    | % blink_msg_end = hrt_absolute_time() + BLINK_MSG_TIME;
    | % rgbled_set_color_and_mode(led_control_s::COLOR_YELLOW, led_control_s::MODE_BLINK_FAST);
    | % 
    | if use_buzzer
    | %     set_tune(tune_control_s::TUNE_ID_NOTIFY_NEUTRAL);
    | end
    | 
    | end % function end
  function tune_mission_ok(use_buzzer):
    | function tune_mission_ok(use_buzzer)
    | 
    | % blink_msg_end = hrt_absolute_time() + BLINK_MSG_TIME;
    | % rgbled_set_color_and_mode(led_control_s::COLOR_GREEN, led_control_s::MODE_BLINK_FAST);
    | % 
    | if use_buzzer
    | %     set_tune(tune_control_s::TUNE_ID_NOTIFY_POSITIVE);
    | end
    | 
    | end % function end
  function geofence_check:
    | function geofence_check
    | 
    | % parameters init
    | persistent geofence_violated_prev
    | persistent geofence_loiter_on
    | persistent geofence_rtl_on
    | persistent geofence_land_on
    | 
    | if isempty(geofence_violated_prev)
    |     geofence_violated_prev = false;
    | end
    | 
    | if isempty(geofence_loiter_on)
    |     geofence_loiter_on = false;
    | end
    | 
    | if isempty(geofence_rtl_on)
    |     geofence_rtl_on = false;
    | end
    | 
    | if isempty(geofence_land_on)
    |     geofence_land_on = false;
    | end
    | 
    | in_low_battery_failsafe = battery_warning_ > PX4_BATTERY_STATUS.BATTERY_WARNING_LOW;
    | 
    | % Geofence actions
    | geofence_action_enabled = (geofence_result.geofence_action ~= PX4_GEOFENCE_RESULT.GF_ACTION_NONE);
    | 
    | if actuator_armed_out_.armed && geofence_action_enabled && ~in_low_battery_failsafe
    | 
    |     switch geofence_result.geofence_action
    | 
    |         case PX4_GEOFENCE_RESULT.GF_ACTION_NONE
    |             % do nothing
    | 
    |         case PX4_GEOFENCE_RESULT.GF_ACTION_WARN
    |             % do nothing, mavlink critical messages are sent by navigator
    | 
    |         case PX4_GEOFENCE_RESULT.GF_ACTION_LOITER
    |             if main_state_transition(PX4_COMMANDER_STATE.MAIN_STATE_AUTO_LOITER) == TRANSITION_CHANGED
    |                 geofence_loiter_on = true;
    |             end
    | 
    |         case PX4_GEOFENCE_RESULT.GF_ACTION_RTL
    |             if main_state_transition(PX4_COMMANDER_STATE.MAIN_STATE_AUTO_RTL) == TRANSITION_CHANGED
    |                 geofence_rtl_on = true;
    |             end
    | 
    |         case PX4_GEOFENCE_RESULT.GF_ACTION_LAND
    |             if main_state_transition(PX4_COMMANDER_STATE.MAIN_STATE_AUTO_LAND) == TRANSITION_CHANGED
    |                 geofence_land_on = true;
    |             end
    | 
    |         case PX4_GEOFENCE_RESULT.GF_ACTION_TERMINATE
    |             sprintf("PX4_WARN, Flight termination because of geofence");
    |             if ~flight_termination_triggered_ && ~lockdown_triggered_
    |                 flight_termination_triggered_ = true;
    |                 sprintf("mavlink_log_critical, Geofence violation! Flight terminated");
    |                 actuator_armed_out_.force_failsafe = true;
    |                 g_status_changed = true;
    |                 % send_parachute_command();
    |             end
    |     end
    | 
    |     geofence_violated_prev = geofence_result.geofence_violated;
    | 
    |     % reset if no longer in LOITER or if manually switched to LOITER
    |     in_loiter_mode = (internal_state_out_.main_state == PX4_COMMANDER_STATE.MAIN_STATE_AUTO_LOITER);
    |     manual_loiter_switch_on = (manual_control_switches.loiter_switch == PX4_MANUAL_CONTROL_SWITCHES.SWITCH_POS_ON);
    | 
    |     if ~in_loiter_mode || manual_loiter_switch_on
    |         geofence_loiter_on = false;
    |     end
    | 
    |     % reset if no longer in RTL or if manually switched to RTL
    |     in_rtl_mode = (internal_state_out_.main_state == PX4_COMMANDER_STATE.MAIN_STATE_AUTO_RTL);
    |     manual_return_switch_on = (manual_control_switches.return_switch == PX4_MANUAL_CONTROL_SWITCHES.SWITCH_POS_ON);
    |     if ~in_rtl_mode || manual_return_switch_on
    |         geofence_rtl_on = false;
    |     end
    | 
    |     % reset if no longer in LAND or if manually switched to LAND
    |     in_land_mode = internal_state_out_.main_state == (PX4_COMMANDER_STATE.MAIN_STATE_AUTO_LAND);
    |     if ~in_land_mode
    |         geofence_land_on = false;
    |     end
    | 
    |     geofence_warning_action_on_ = geofence_warning_action_on_ || ...
    |         (geofence_loiter_on || geofence_rtl_on || geofence_land_on);
    | 
    | else
    |     %% No geofence checks, reset flags
    |     geofence_loiter_on = false;
    |     geofence_rtl_on = false;
    |     geofence_land_on = false;
    |     geofence_violated_prev = false;
    |     geofence_warning_action_on_ = false;
    | end
    | 
    | end % function end
  function manual_control_input_handling:
    | function manual_control_input_handling()
    | 
    | rc_allowed = ~vehicle_status_flags_out_.rc_input_blocked;
    | 
    | %% manual control update
    | if manual_control_update()
    | 
    |     %% handle the case where RC signal was regained
    |     if ~vehicle_status_flags_out_.rc_signal_found_once
    |         vehicle_status_flags_out_.rc_signal_found_once = true;
    |         set_health_flags(SUBSYSTEM_TYPE_RCRECEIVER, true, true, vehicle_status_flags_out_.rc_calibration_valid, vehicle_status_out_);
    |         g_status_changed = true;
    |     else
    |         if vehicle_status_out_.rc_signal_lost
    |             if rc_signal_lost_timestamp > 0
    |                 sprintf("mavlink_log_info, Manual control regained after %fs", single(uint64(getSimulationTime*1e+6) - rc_signal_lost_timestamp) * 1e-6);
    |             end
    |             set_health_flags(SUBSYSTEM_TYPE_RCRECEIVER, true, true, vehicle_status_flags_out_.rc_calibration_valid, vehicle_status_out_);
    |             g_status_changed = true;
    |         end
    |     end
    | 
    |     vehicle_status_out_.rc_signal_lost = false;
    | 
    |     %% inform the user
    |     rc_arming_enabled = (vehicle_status_out_.rc_input_mode ~= PX4_VEHICLE_STATUS.RC_IN_MODE_OFF);
    |     if rc_arming_enabled
    |         if manual_control_wantsDisarm()
    |             send(EVT_DISARM_RC_STICK, arming_state_transition);
    |         end
    | 
    |         if manual_control_wantsArm()
    |             if control_mode_out_.flag_control_manual_enabled
    |                 send(EVT_ARM_RC_STICK, arming_state_transition);
    |             else
    |                 sprintf("mavlink_log_critical, Not arming! Switch to a manual mode first");
    |                 % tune_negative(true);
    |             end
    |         end
    |     end
    | end
    | 
    | end % function end
    | 
    | 
    | 
    | %% manual_control_update
    | function ret = manual_control_update()
    | 
    | updated = false;
    | 
    | if hasChanged(manual_control_setpoint.timestamp)
    |     last_manual_control_setpoint = manual_control_setpoint;
    |     updated = true;
    | end
    | 
    | rc_available = rc_allowed && ...
    |     manual_control_setpoint.timestamp ~= 0 && ...
    |     ((uint64(getSimulationTime*1e+6) - manual_control_setpoint.timestamp) < (COM_RC_LOSS_T*1e+6));
    | 
    | ret = updated && rc_available;
    | 
    | end % function manual_control_update() end
    | 
    | %% manual_control_wantsDisarm
    | function ret = manual_control_wantsDisarm()
    | 
    | ret = false;
    | 
    | use_stick  = (manual_control_switches.arm_switch == PX4_MANUAL_CONTROL_SWITCHES.SWITCH_POS_NONE);
    | use_button = (~use_stick && COM_ARM_SWISBTN);
    | use_switch = (~use_stick && ~use_button);
    | armed      = (vehicle_status_out_.arming_state == PX4_VEHICLE_STATUS.ARMING_STATE_ARMED);
    | 
    | stick_in_lower_left = use_stick && (last_manual_control_setpoint.z < 0.1) && (manual_control_setpoint.r < -0.9);
    | 
    | arm_button_pressed = (manual_control_switches.arm_switch == PX4_MANUAL_CONTROL_SWITCHES.SWITCH_POS_ON) && use_button;
    | 
    | arm_switch_to_disarm_transition = use_switch && ...
    |     (last_manual_control_switches_arm_switch == PX4_MANUAL_CONTROL_SWITCHES.SWITCH_POS_ON) && ...
    |     (manual_control_switches.arm_switch == PX4_MANUAL_CONTROL_SWITCHES.SWITCH_POS_OFF);
    | 
    | mc_manual_thrust_mode = (vehicle_status_out_.vehicle_type == PX4_VEHICLE_STATUS.VEHICLE_TYPE_ROTARY_WING) && ...
    |     control_mode_out_.flag_control_manual_enabled && ...
    |     ~control_mode_out_.flag_control_climb_rate_enabled;
    | 
    | if armed && (land_detector.landed || mc_manual_thrust_mode) && (stick_in_lower_left || arm_button_pressed || arm_switch_to_disarm_transition)
    | 
    |     stick_disarm_hysteresis_state = true;
    | 
    |     if (uint64(getSimulationTime*1e+6) - last_change_disarm_time) > COM_RC_ARM_HYST
    |         last_change_disarm_time = uint64(getSimulationTime*1e+6);
    |     end
    | 
    |     disarm_trigger = ~last_stick_disarm_hysteresis_state && stick_disarm_hysteresis_state;
    | 
    |     if disarm_trigger || arm_switch_to_disarm_transition
    |         ret = true;
    |     end
    | else
    | 
    |     stick_disarm_hysteresis_state = false;
    | end
    | 
    | last_stick_disarm_hysteresis_state = stick_disarm_hysteresis_state;
    | 
    | end % function manual_control_wantsDisarm() end
    | 
    | %% manual_control_wantsDisarm
    | function ret = manual_control_wantsArm()
    | 
    | ret = false;
    | 
    | use_stick  = (manual_control_switches.arm_switch == PX4_MANUAL_CONTROL_SWITCHES.SWITCH_POS_NONE);
    | use_button = (~use_stick && COM_ARM_SWISBTN);
    | use_switch = (~use_stick && ~use_button);
    | armed      = (vehicle_status_out_.arming_state == PX4_VEHICLE_STATUS.ARMING_STATE_ARMED);
    | 
    | stick_in_lower_right = use_stick && (last_manual_control_setpoint.z < 0.1) && (manual_control_setpoint.r > -0.9);
    | 
    | arm_button_pressed = (manual_control_switches.arm_switch == PX4_MANUAL_CONTROL_SWITCHES.SWITCH_POS_ON) && use_button;
    | 
    | arm_switch_to_arm_transition = use_switch && ...
    |     (last_manual_control_switches_arm_switch == PX4_MANUAL_CONTROL_SWITCHES.SWITCH_POS_OFF) && ...
    |     (manual_control_switches.arm_switch == PX4_MANUAL_CONTROL_SWITCHES.SWITCH_POS_ON);
    | 
    | if armed && (stick_in_lower_right || arm_button_pressed || arm_switch_to_arm_transition)
    | 
    |     stick_arm_hysteresis_state = true;
    | 
    |     if (uint64(getSimulationTime*1e+6) - last_change_arm_time) > COM_RC_ARM_HYST
    |         last_change_arm_time = uint64(getSimulationTime*1e+6);
    |     end
    | 
    |     arm_trigger = ~last_stick_disarm_hysteresis_state && stick_arm_hysteresis_state;
    | 
    |     if arm_trigger || arm_switch_to_arm_transition
    |         ret = true;
    |     end
    | else
    | 
    |     stick_arm_hysteresis_state = false;
    | end
    | 
    | last_stick_disarm_hysteresis_state = stick_arm_hysteresis_state;
    | 
    | end % fuction manual_control_wantsArm() end
  function check_engine_failure_for_fixed_wing:
    | function check_engine_failure_for_fixed_wing()
    | 
    | throttle = actuator_controls.control(PX4_ACTUATOR_CONTROLS.INDEX_THROTTLE);
    | current2throttle = battery_current_ / throttle;
    | 
    | if (( (throttle > COM_EF_THROT) && (current2throttle < COM_EF_C2T)) || vehicle_status_out_.engine_failure)
    |     
    |     elapsed = (uint64(getSimulationTime*1e+6) - timestamp_engine_healthy) / 1e+6;
    |     
    |     % potential failure, measure time
    |     if ((timestamp_engine_healthy > 0) && (elapsed > COM_EF_TIME) && ~vehicle_status_out_.engine_failure)
    |         vehicle_status_out_.engine_failure = true;
    |         g_status_changed = true;
    |         sprintf("PX4_ERR, Engine Failure")
    |         set_health_flags(SUBSYSTEM_TYPE_MOTORCONTROL, true, true, false, vehicle_status_out_);
    |     end
    | end
    | 
    | 
    | end
  function reset_failure_flags:
    | function reset_failure_flags
    | 
    | % no failure reset flag
    | timestamp_engine_healthy = uint64(getSimulationTime * 1e+6);
    | 
    | if vehicle_status_out_.engine_failure
    |     vehicle_status_out_.engine_failure = false;
    |     g_status_changed = true;
    | end
    | 
    | end
  function set_home_lpos_valid:
    | function set_home_lpos_valid()
    | 
    | % distance from home
    | distance = -1.0;
    | home_dist_xy = -1.0;
    | home_dist_z = -1.0;
    | 
    | [distance, home_dist_xy, home_dist_z] = mavlink_wpm_distance_to_point_local(home_position.x, home_position.y, home_position.z, local_position.x, local_position.y, local_position.z);
    | 
    | if (home_dist_xy > local_position.eph * 2.0) || (home_dist_z > local_position.epv * 2.0)
    |     % update when disarmed, landed and moved away from current home position
    |     set_home_position();
    | end
    | 
    | end
  function set_home_lpos_invalid:
    | function set_home_lpos_invalid()
    | 
    | 
    | 
    | 
    | end
  function reset_posvel_validity:
    | function reset_posvel_validity()
    | 
    | % reset all the check probation times back to the minimum value
    | % 将所有检查试用时间重置为最小值
    | gpos_probation_time_us_ = POSVEL_PROBATION_MIN;
    | lpos_probation_time_us_ = POSVEL_PROBATION_MIN;
    | lvel_probation_time_us_ = POSVEL_PROBATION_MIN;
    | 
    | % recheck validity
    | % 重新检查有效性
    | UpdateEstimateValidity();
    | 
    | end
  function set_custom_home_position(home_lat, home_lon, home_alt):
    | function set_custom_home_position(home_lat, home_lon, home_alt)
    | 
    | if local_position.xy_global && local_position.z_global
    |     % use specified position
    |     home_position_out_.timestamp = uint64(getSimulationTime() * 1e+6);
    |     fillGlobalHomePos(home_position_out_, home_lat, home_lon, home_alt);
    |     home_position_out_.manual_home = true;
    |     
    |     % update local projection reference including altitude
    |     ref_pos = map_projection_init(local_position.ref_lat, local_position.ref_lon);
    |     [home_x, home_y] = map_projection_project(ref_pos, home_lat, home_lon);
    |     home_z = -(home_alt - local_position.ref_alt);
    |     % fillLocalHomePos(home_pos, local_pos);
    |     home_position_out_.x = home_x;
    |     home_position_out_.y = home_y;
    |     home_position_out_.z = home_z;
    |     home_position_out_.yaw = single(0.0);
    |     
    |     % mark home position as set
    |     vehicle_status_flags_out_.condition_home_position_valid = true; % _home_pub.update(home);
    |     cmd_result = uint8(PX4_VEHICLE_COMMAND.VEHICLE_CMD_RESULT_ACCEPTED);
    | else
    |     cmd_result = uint8(PX4_VEHICLE_COMMAND.VEHICLE_CMD_RESULT_TEMPORARILY_REJECTED);
    | end
    | 
    | end
  function fixed_mag_cal_yaw:
    | function fixed_mag_cal_yaw
    | 
    | % parameter 1: Heading   (degrees)
    | % parameter 3: Latitude  (degrees)
    | % parameter 4: Longitude (degrees)
    | 
    | % assume vehicle pointing north (0 degrees) if heading isn't specified
    | if isfinite(cmd.param1)
    |     heading_radians = single(deg2rad(round(cmd.param1)));
    | else
    |     heading_radians = single(0.0);
    | end
    | 
    | latitude = nan;
    | longitude = nan;
    | 
    | if isfinite(cmd.param3) && isfinite(cmd.param4)
    |     % invalid if both lat & lon are 0 (current mavlink spec)
    |     if ((abs(cmd.param3) > 0) && (abs(cmd.param4) > 0))
    |         latitude = cmd.param3;
    |         longitude = cmd.param4;
    |     end
    | end
    | 
    | vehicle_status_flags_out_.condition_calibration_enabled = true;
    | % _worker_thread.setMagQuickData(heading_radians, latitude, longitude);
    | % _worker_thread.startTask(WorkerThread::Request::MagCalibrationQuick);
    | 
    | end
  function set_health_flags_healthy(subsystem_type, healthy, status):
    | function set_health_flags_healthy(subsystem_type, healthy, status)
    | 
    | set_health_flags(subsystem_type, ...
    |     bitand(status.onboard_control_sensors_present, subsystem_type), ...
    |     bitand(status.onboard_control_sensors_enabled, subsystem_type), ...
    |     healthy, ...
    |     status);
    | 
    | end
  function set_health_flags(subsystem_type, present, enabled, ok, status):
    | function set_health_flags(subsystem_type, present, enabled, ok, status)
    | 
    | sprintf("set_health_flags: Type %llu pres=%u enabl=%u ok=%u");
    | 
    | if (present)
    |     status.onboard_control_sensors_present = bitor(status.onboard_control_sensors_present, subsystem_type);
    | else
    |     status.onboard_control_sensors_present = bitand(status.onboard_control_sensors_present, bitcmp(subsystem_type));
    | end
    | 
    | if (enabled)
    |     status.onboard_control_sensors_enabled = bitor((status.onboard_control_sensors_enabled), subsystem_type);
    | else
    |     status.onboard_control_sensors_enabled = bitand((status.onboard_control_sensors_enabled), bitcmp(subsystem_type));
    | end
    | 
    | if (ok)
    |     status.onboard_control_sensors_health = bitor(status.onboard_control_sensors_health, subsystem_type);
    | else
    |     status.onboard_control_sensors_health = bitand(status.onboard_control_sensors_health, bitcmp(subsystem_type));
    | end
    | 
    | end
  function UpdateEstimateValidity:
    | % Horizontal position error threshold.
    | % This is the horizontal position error (EPH) threshold that will trigger a failsafe. The default is appropriate for a multicopter. Can be increased for a fixed-wing.
    | % @unit m
    | % @group Commander
    | % PARAM_DEFINE_FLOAT(COM_POS_FS_EPH, 5);
    |  function UpdateEstimateValidity()
    | 
    | lpos_eph_threshold_adj = COM_POS_FS_EPH;
    | 
    | % relax local position eph threshold in operator controlled position mode
    | % 在位置模式下操作时，放宽local_pos的阈值
    | % // relax local position eph threshold in operator controlled position mode
    | % if (_internal_state.main_state == commander_state_s::MAIN_STATE_POSCTL &&
    | %     ((_status.nav_state == vehicle_status_s::NAVIGATION_STATE_ALTCTL)
    | %      || (_status.nav_state == vehicle_status_s::NAVIGATION_STATE_POSCTL))) {
    | % 
    | %     // Set the allowable position uncertainty based on combination of flight and estimator state
    | %     // When we are in a operator demanded position control mode and are solely reliant on optical flow, do not check position error because it will gradually increase throughout flight and the operator will compensate for the drift
    | %     const bool reliant_on_opt_flow = ((status.control_mode_flags & (1 << estimator_status_s::CS_OPT_FLOW))
    | %                       && !(status.control_mode_flags & (1 << estimator_status_s::CS_GPS))
    | %                       && !(status.control_mode_flags & (1 << estimator_status_s::CS_EV_POS)));
    | % 
    | %     if (reliant_on_opt_flow) {
    | %         lpos_eph_threshold_adj = INFINITY;
    | %     }
    | % }
    | 
    | % 此部分需要完成估计器检查那段代码
    | % vehicle_status_flags_out_.condition_global_position_valid = check_posvel_validity(lpos.xy_valid && !_nav_test_failed, gpos.eph, _param_com_pos_fs_eph.get(), gpos.timestamp,
    | % 				      &_last_gpos_fail_time_us, &_gpos_probation_time_us, _status_flags.condition_global_position_valid);
    | % 
    | % vehicle_status_flags_out_.condition_local_position_valid = check_posvel_validity(lpos.xy_valid && !_nav_test_failed, lpos.eph, lpos_eph_threshold_adj, lpos.timestamp,
    | % 				      &_last_lpos_fail_time_us, &_lpos_probation_time_us, _status_flags.condition_local_position_valid);
    | % 
    | % vehicle_status_flags_out_.condition_local_velocity_valid = check_posvel_validity(lpos.v_xy_valid && !_nav_test_failed, lpos.evh, _param_com_vel_fs_evh.get(), lpos.timestamp,
    | % 				      &_last_lvel_fail_time_us, &_lvel_probation_time_us, _status_flags.condition_local_velocity_valid);
    |                       
    | end
  function setHomePosValid:
    | function setHomePosValid()
    | 
    | % 	// play tune first time we initialize HOME
    | % 	if (!_status_flags.condition_home_position_valid) {
    | % 		tune_home_set(true);
    | % 	}
    | 
    | % mark home position as set
    | status_flags_out_.condition_home_position_valid = true;
    | 
    | end
  function ret = check_posvel_validity(data_valid, data_accuracy, ...:
    | function ret = check_posvel_validity(data_valid, data_accuracy, ...
    |     required_accuracy, data_timestamp_us, ...
    |     last_fail_time_us, probation_time_us, was_valid)
    | 
    | ret = was_valid;
    | 
    | % constrain probation times
    | if land_detector.landed
    |     probation_time_us = POSVEL_PROBATION_MIN;
    | end
    | 
    | data_stale = ((uint64(getSimulationTime*1e+6) - data_timestamp_us) > COM_POS_FS_DELAY*1e+6) || (data_timestamp_us == 0);
    | 
    | if was_valid
    |     req_accuracy = required_accuracy * 2.5;
    | else
    |     req_accuracy = required_accuracy;
    | end
    | 
    | level_check_pass = data_valid && ~data_stale && (data_accuracy < req_accuracy);
    | 
    | % Check accuracy with hysteresis in both test level and time
    | if level_check_pass
    |     
    |     if was_valid
    |         % still valid, continue to decrease probation time
    |         probation_time_new = probation_time_us - (uint64(getSimulationTime*1e+6) - last_fail_time_us);
    |         probation_time_us = constrain(probation_time_new, POSVEL_PROBATION_MIN, POSVEL_PROBATION_MAX);
    |     else
    |         % check if probation period has elapsed
    |         if (uint64(getSimulationTime*1e+6) - last_fail_time_us) > probation_time_us
    |             ret = true;
    |         else
    |             % level check failed
    |             if was_valid
    |                 % FAILURE~ no longer valid
    |                 ret = false;
    |             else
    |                 % failed again, increase probation time
    |                 probation_time_new = probation_time_us + (uint64(getSimulationTime*1e+6) - last_fail_time_us) * uint64(COM_POS_FS_GAIN);
    |                 probation_time_us = constrain(probation_time_new, POSVEL_PROBATION_MIN, POSVEL_PROBATION_MAX);
    |             end
    |             last_fail_time_us = uint64(getSimulationTime)*1e+6;
    |         end
    |         
    |         if was_valid ~= ret
    |             g_status_changed = true;
    |         end
    |     end
    |     
    |     ret = ret;
    |     
    | end
    | 
    | end % function end
  function arm_state_in_init_tans_to_standby:
    | function arm_state_in_init_tans_to_standby()
    | 
    | persistent last_preflight_check;
    | 
    | if isempty(last_preflight_check)
    |     last_preflight_check = uint64(0);
    | end
    | 
    | if vehicle_status_flags_out_.condition_system_sensors_initialized && ...
    |         (last_preflight_check == 0 || (uint64(getSimulationTime*1e+6) - last_preflight_check > 1e+6))
    |     
    | %     vehicle_status_flags_out_.condition_system_sensors_initialized = PreFlightCheck::preflightCheck(mavlink_log_pub, status,
    | %     status_flags, false, status.arming_state != vehicle_status_s::ARMING_STATE_ARMED,
    | %     time_since_boot);
    |     
    |     last_preflight_check = uint64(getSimulationTime*1e+6);
    |     
    | end
    | 
    | end
  function enable_failsafe(reason):
    | function enable_failsafe(reason)
    | 
    | % Enable failsafe and report to user
    | if (~old_failsafe && vehicle_status_out_.arming_state == PX4_VEHICLE_STATUS.ARMING_STATE_ARMED)
    |     
    |     % make sure intermittent failsafes don't lead to infinite delay by not constantly reseting the timestamp
    |     if ((vehicle_status_out_.failsafe_timestamp == 0 || uint64(getSimulationTime*1e+6) - (vehicle_status_out_.failsafe_timestamp) > 30*1e+6))
    |         vehicle_status_out_.failsafe_timestamp = uint64(getSimulationTime*1e+6);
    |     end
    |     
    |     sprintf("mavlink_log_critical, Failsafe enabled, %s", reason)
    |     vehicle_status_out_.failsafe = true;
    |     
    | end
    | 
    | end
  function set_link_loss_nav_state(link_loss_act, ll_delay):
    | function set_link_loss_nav_state(link_loss_act, ll_delay)
    | 
    | if (uint64(getSimulationTime*1e+6) - vehicle_status_out_.failsafe_timestamp) < (ll_delay * 1e+6) && ...
    |         (link_loss_act ~= PX4_LINK_LOSS_ACTIONS.DISABLED)
    |     % delay failsafe reaction by trying to hold position if configured
    |     link_loss_act = int32(PX4_LINK_LOSS_ACTIONS.AUTO_LOITER);
    | end
    | 
    | % do the best you can according to the action set
    | switch link_loss_act
    |     
    |     case PX4_LINK_LOSS_ACTIONS.DISABLED
    |         % If datalink loss failsafe is disabled then no action must be taken.
    |         
    |     case PX4_LINK_LOSS_ACTIONS.AUTO_RTL
    |         if vehicle_status_flags_out_.condition_global_position_valid && status_flags.condition_home_position_valid
    |             main_state_transition(PX4_COMMANDER_STATE.MAIN_STATE_AUTO_RTL);
    |             vehicle_status_out_.nav_state = uint8(PX4_VEHICLE_STATUS.NAVIGATION_STATE_AUTO_RTL);
    |             return
    |         end
    |         
    |     case PX4_LINK_LOSS_ACTIONS.AUTO_LOITER
    |         % FALLTHROUGH
    |         if vehicle_status_flags_out_.condition_global_position_valid
    |             vehicle_status_out_.nav_state = uint8(PX4_VEHICLE_STATUS.NAVIGATION_STATE_AUTO_LOITER);
    |             return
    |         end
    |         
    |     case PX4_LINK_LOSS_ACTIONS.AUTO_LAND
    |         % FALLTHROUGH
    |         if vehicle_status_flags_out_.condition_global_position_valid
    |             vehicle_status_out_.nav_state = uint8(PX4_VEHICLE_STATUS.NAVIGATION_STATE_AUTO_LAND);
    |             return
    |         else
    |             if vehicle_status_out_.vehicle_type == PX4_VEHICLE_STATUS.VEHICLE_TYPE_ROTARY_WING
    |                 if vehicle_status_flags_out_.condition_local_position_valid
    |                     vehicle_status_out_.nav_state = uint8(PX4_VEHICLE_STATUS.NAVIGATION_STATE_AUTO_LAND);
    |                     return
    |                 elseif vehicle_status_flags_out_.condition_local_altitude_valid
    |                     vehicle_status_out_.nav_state = uint8(PX4_VEHICLE_STATUS.NAVIGATION_STATE_DESCEND);
    |                     return
    |                 end
    |             else
    |                 % TODO: FW position controller doesn't run without condition_global_position_valid
    |                 vehicle_status_out_.nav_state = uint8(PX4_VEHICLE_STATUS.NAVIGATION_STATE_AUTO_LANDGPSFAIL);
    |                 return
    |             end
    |         end
    |         
    |     case PX4_LINK_LOSS_ACTIONS.TERMINATE
    |         % FALLTHROUGH
    |         vehicle_status_out_.nav_state = uint8(PX4_VEHICLE_STATUS.NAVIGATION_STATE_TERMINATION);
    |         actuator_armed_out_.force_failsafe = true;
    |         
    |     case PX4_LINK_LOSS_ACTIONS.LOCKDOWN
    |         actuator_armed_out_.lockdown = true;
    |         
    | end
    | 
    | end
  function fallback_required = check_invalid_pos_nav_state(use_rc, using_global_pos):
    | % Checks the validty of position data against the requirements of the current navigation
    | % mode and switches mode if position data required is not available.
    | function fallback_required = check_invalid_pos_nav_state(use_rc, using_global_pos)
    | 
    | fallback_required = false;
    | 
    | if using_global_pos && vehicle_status_flags_out_.condition_global_position_valid
    |     fallback_required = true;
    | elseif ~using_global_pos && (~vehicle_status_flags_out_.condition_local_position_valid || ~vehicle_status_flags_out_.condition_local_velocity_valid)
    |     fallback_required = true;
    | end
    | 
    | if fallback_required
    |     
    |     %% use rc
    |     if use_rc
    |         % fallback to a mode that gives the operator stick control
    |         if (vehicle_status_out_.vehicle_type == PX4_VEHICLE_STATUS.VEHICLE_TYPE_ROTARY_WING) && vehicle_status_flags_out_.condition_local_position_valid
    |             vehicle_status_out_.nav_state = uint8(PX4_VEHICLE_STATUS.NAVIGATION_STATE_POSCTL);
    |         elseif vehicle_status_flags_out_.condition_local_altitude_valid
    |             vehicle_status_out_.nav_state = uint8(PX4_VEHICLE_STATUS.NAVIGATION_STATE_ALTCTL);
    |         else
    |             vehicle_status_out_.nav_state = uint8(PX4_VEHICLE_STATUS.NAVIGATION_STATE_STAB);
    |         end
    |     else
    |         % go into a descent that does not require stick control
    |         if vehicle_status_flags_out_.condition_local_position_valid
    |             vehicle_status_out_.nav_state = uint8(PX4_VEHICLE_STATUS.NAVIGATION_STATE_AUTO_LAND);
    |         elseif vehicle_status_flags_out_.condition_local_altitude_valid
    |             if vehicle_status_out_.vehicle_type == PX4_VEHICLE_STATUS.VEHICLE_TYPE_ROTARY_WING
    |                 vehicle_status_out_.nav_state = uint8(PX4_VEHICLE_STATUS.NAVIGATION_STATE_DESCEND);
    |             else
    |                 % TODO: FW position controller doesn't run without condition_global_position_valid
    |                 vehicle_status_out_.nav_state = uint8(PX4_VEHICLE_STATUS.NAVIGATION_STATE_AUTO_LANDGPSFAIL);
    |             end
    |         else
    |             vehicle_status_out_.nav_state = uint8(PX4_VEHICLE_STATUS.NAVIGATION_STATE_TERMINATION);
    |         end
    |     end
    |     
    |     %% use global pos
    |     if using_global_pos
    |         set_navigation_state.enable_failsafe("no global position");
    |     else
    |         set_navigation_state.enable_failsafe("no local position");
    |     end
    |     
    | end
    | 
    | end
  function set_offboard_loss_nav_state(offboard_loss_act):
    | function set_offboard_loss_nav_state(offboard_loss_act)
    | 
    | switch offboard_loss_act
    |     
    |     case PX4_OFFBOARD_LOSS_ACTIONS.DISABLED
    |         % If offboard loss failsafe is disabled then no action must be taken.
    |         return
    |         
    |     case PX4_OFFBOARD_LOSS_ACTIONS.TERMINATE
    |         vehicle_status_out_.nav_state = uint8(PX4_VEHICLE_STATUS.NAVIGATION_STATE_TERMINATION);
    |         actuator_armed_out_.force_failsafe = true;
    |         return
    |         
    |     case PX4_OFFBOARD_LOSS_ACTIONS.LOCKDOWN
    |         actuator_armed_out_.lockdown = true;
    |         return
    |         
    |     case PX4_OFFBOARD_LOSS_ACTIONS.AUTO_RTL
    |         if status_flags.condition_global_position_valid && status_flags.condition_home_position_valid
    |             vehicle_status_out_.nav_state = uint8(PX4_VEHICLE_STATUS.NAVIGATION_STATE_AUTO_RTL);
    |             return
    |         end
    |         
    |     case PX4_OFFBOARD_LOSS_ACTIONS.AUTO_LOITER
    |         % FALLTHROUGH
    |         if vehicle_status_flags_out_.condition_global_position_valid
    |             vehicle_status_out_.nav_state = uint8(PX4_VEHICLE_STATUS.NAVIGATION_STATE_AUTO_LOITER);
    |             return;
    |         end
    |         
    |     case PX4_OFFBOARD_LOSS_ACTIONS.AUTO_LAND
    |         % FALLTHROUGH
    |         if vehicle_status_flags_out_.condition_global_position_valid
    |             vehicle_status_out_.nav_state = uint8(PX4_VEHICLE_STATUS.NAVIGATION_STATE_AUTO_LAND);
    |             return
    |         end
    |         
    | end
    | 
    | % If none of the above worked, try to mitigate
    | if vehicle_status_flags_out_.condition_local_altitude_valid
    |     if (vehicle_status_out_.vehicle_type == PX4_VEHICLE_STATUS.VEHICLE_TYPE_ROTARY_WING)
    |         vehicle_status_out_.nav_state = uint8(PX4_VEHICLE_STATUS.NAVIGATION_STATE_DESCEND);
    |     else
    |         % TODO: FW position controller doesn't run without condition_global_position_valid
    |         vehicle_status_out_.nav_state = uint8(PX4_VEHICLE_STATUS.NAVIGATION_STATE_AUTO_LANDGPSFAIL);
    |     end
    | else
    |     vehicle_status_out_.nav_state = uint8(PX4_VEHICLE_STATUS.NAVIGATION_STATE_TERMINATION);
    | end
    | 
    | end
  function set_offboard_loss_rc_nav_state(offboard_loss_rc_act):
    | function set_offboard_loss_rc_nav_state(offboard_loss_rc_act)
    | 
    | switch offboard_loss_rc_act
    |     
    |     case PX4_OFFBOARD_LOSS_RC_ACTIONS.DISABLED
    |         % If offboard loss failsafe is disabled then no action must be taken.
    |         return
    |         
    |     case PX4_OFFBOARD_LOSS_RC_ACTIONS.TERMINATE
    |         vehicle_status_out_.nav_state = uint8(PX4_VEHICLE_STATUS.NAVIGATION_STATE_TERMINATION);
    |         actuator_armed_out_.force_failsafe = true;
    |         return
    |         
    |     case PX4_OFFBOARD_LOSS_RC_ACTIONS.LOCKDOWN
    |         actuator_armed_out_.lockdown = true;
    |         return
    |         
    |     case PX4_OFFBOARD_LOSS_RC_ACTIONS.MANUAL_POSITION
    |         if vehicle_status_out_.vehicle_type == PX4_VEHICLE_STATUS.VEHICLE_TYPE_ROTARY_WING && ...
    |                 vehicle_status_flags_out_.condition_local_position_valid
    |             vehicle_status_out_.nav_state = uint8(PX4_VEHICLE_STATUS.NAVIGATION_STATE_POSCTL);
    |             return
    |         elseif vehicle_status_flags_out_.condition_global_position_valid
    |             vehicle_status_out_.nav_state = uint8(PX4_VEHICLE_STATUS.NAVIGATION_STATE_POSCTL);
    |             return
    |         end
    |         
    |         
    |     case PX4_OFFBOARD_LOSS_RC_ACTIONS.MANUAL_ALTITUDE
    |         % FALLTHROUGH
    |         if vehicle_status_flags_out_.condition_local_altitude_valid
    |             vehicle_status_out_.nav_state = uint8(PX4_VEHICLE_STATUS.NAVIGATION_STATE_ALTCTL);
    |             return
    |         end
    |         
    |     case PX4_OFFBOARD_LOSS_RC_ACTIONS.MANUAL_ATTITUDE
    |         % FALLTHROUGH
    |         vehicle_status_out_.nav_state = uint8(PX4_VEHICLE_STATUS.NAVIGATION_STATE_MANUAL);
    |         return
    |         
    |     case PX4_OFFBOARD_LOSS_RC_ACTIONS.AUTO_RTL
    |         if vehicle_status_flags_out_.condition_global_position_valid && status_flags.condition_home_position_valid
    |             vehicle_status_out_.nav_state = uint8(PX4_VEHICLE_STATUS.NAVIGATION_STATE_AUTO_RTL);
    |             return
    |         end
    |         
    |         
    |     case PX4_OFFBOARD_LOSS_RC_ACTIONS.AUTO_LOITER
    |         % FALLTHROUGH
    |         if vehicle_status_flags_out_.condition_global_position_valid
    |             vehicle_status_out_.nav_state = uint8(PX4_VEHICLE_STATUS.NAVIGATION_STATE_AUTO_LOITER);
    |             return
    |         end
    |         
    |     case PX4_OFFBOARD_LOSS_RC_ACTIONS.AUTO_LAND
    |         % FALLTHROUGH
    |         if vehicle_status_flags_out_.condition_global_position_valid
    |             vehicle_status_out_.nav_state = uint8(PX4_VEHICLE_STATUS.NAVIGATION_STATE_AUTO_LAND);
    |             return
    |         end
    |         
    | end
    | 
    | % If none of the above worked, try to mitigate
    | if vehicle_status_flags_out_.condition_local_altitude_valid
    |     %TODO: Add case for rover
    |     if vehicle_status_out_.vehicle_type == PX4_VEHICLE_STATUS.VEHICLE_TYPE_ROTARY_WING
    |         vehicle_status_out_.nav_state = uint8(PX4_VEHICLE_STATUS.NAVIGATION_STATE_DESCEND);
    |     else
    |         % TODO: FW position controller doesn't run without condition_global_position_valid
    |         vehicle_status_out_.nav_state = uint8(PX4_VEHICLE_STATUS.NAVIGATION_STATE_AUTO_LANDGPSFAIL);
    |     end
    | else
    |     vehicle_status_out_.nav_state = uint8(PX4_VEHICLE_STATUS.NAVIGATION_STATE_TERMINATION);
    | end
    | 
    | end
  function ret = set_home_position:
    | function ret = set_home_position()
    | 
    | % Need global and local position fix to be able to set home
    | % but already set the home position in local coordinates if available
    | % in case the global position is only valid after takeoff
    | if (vehicle_status_flags_out_.condition_local_position_valid)
    |     
    |     home_position_out_.timestamp = uint64(getSimulationTime * 1e+6);
    |     home_position_out_.manual_home = false;
    |     fillLocalHomePos(home_position_out_, local_position);
    |     
    |     if (vehicle_status_flags_out_.condition_global_position_valid)
    |         
    |         % Ensure that the GPS accuracy is good enough for intializing home
    |         if (isGPosGoodForInitializingHomePos(global_position))
    |             fillGlobalHomePos(home_position_out_, global_position.lat, global_position.lon, global_position.alt);
    |             setHomePosValid();
    |         end
    |     end
    |     
    | end
    | 
    | ret = vehicle_status_flags_out_.condition_home_position_valid;
    | 
    | end
  function ret = set_in_air_home_position:
    | % 函数功能：
    | % 允许在飞机起飞后设置home点位置；
    | % 如果参数COM_HOME_IN_AIR设置为true，飞机可以在起飞后设置其home点位置；
    | % 如果一个local_pos估计是准确的，则反向计算真正的home点位置；
    | % 如果没有有效的local_pos，则将home点设置为当前位置。
    | % PARAM_DEFINE_INT32(COM_HOME_IN_AIR, 0);
    | function ret = set_in_air_home_position()
    | 
    | if (vehicle_status_flags_out_.condition_local_position_valid && ...
    |         vehicle_status_flags_out_.condition_global_position_valid)
    |     
    |     % Ensure that the GPS accuracy is good enough for intializing home
    |     if (isGPosGoodForInitializingHomePos(global_position))
    |         
    |         home_position_out_.timestamp = uint64(getSimulationTime * 1e+6);
    |         
    |         if (home_position_out_.valid_lpos)
    |             % Back-compute lon, lat and alt of home position given the home
    |             % and current positions in local frame
    |             ref_pos = map_projection_init(global_position.lat, global_position.lon);
    |             [ret, home_lat, home_lon] = map_projection_reproject(ref_pos, home_position.x - local_position.x, home_position.y - local_position.y);
    |             home_alt = single(global_position.alt + home_position.z);
    |             fillGlobalHomePos(home_position, home_lat, home_lon, home_alt);
    |         else
    |             % Home position in local frame is unknowm, set
    |             % home as current position
    |             fillLocalHomePos(home_position_out_, local_position);
    |             fillGlobalHomePos(home_position_out_, global_position.lon, global_position.lat, global_position.alt);
    |         end
    |         
    |         setHomePosValid();
    |         
    |     end
    | end
    | 
    | ret = vehicle_status_flags_out_.condition_home_position_valid;
    | 
    | end
  function fillGlobalHomePos(home_pos, lat, lon, alt):
    | function fillGlobalHomePos(home_pos, lat, lon, alt)
    | 
    | home_pos.lat = lat;
    | home_pos.lon = lon;
    | home_pos.valid_hpos = true;
    | home_pos.alt = alt;
    | home_pos.valid_alt = true;
    | 
    | end
  function fillLocalHomePos(home_pos, local_pos):
    | function fillLocalHomePos(home_pos, local_pos)
    | 
    | home_pos.x = local_pos.x;
    | home_pos.y = local_pos.y;
    | home_pos.z = local_pos.z;
    | home_pos.valid_lpos = true;
    | home_pos.yaw = local_pos.heading;
    | 
    | end
  function ret = isGPosGoodForInitializingHomePos(gpos):
    | function ret = isGPosGoodForInitializingHomePos(gpos)
    | 
    | ret = (gpos.eph <= COM_HOME_H_T) && (gpos.epv <= COM_HOME_V_T);
    | 
    | end
  function answer_command(cmd_in, result):
    | function answer_command(cmd_in, result)
    | 
    | switch result
    |     case uint8(PX4_VEHICLE_COMMAND.VEHICLE_CMD_RESULT_ACCEPTED)
    |         
    |     case uint8(PX4_VEHICLE_COMMAND.VEHICLE_CMD_RESULT_DENIED)
    | %         tune_negative(true);
    |         
    |     case uint8(PX4_VEHICLE_COMMAND.VEHICLE_CMD_RESULT_FAILED)
    | %         tune_negative(true);
    |         
    |     case uint8(PX4_VEHICLE_COMMAND.VEHICLE_CMD_RESULT_TEMPORARILY_REJECTED)
    | %         tune_negative(true);
    |         
    |     case uint8(PX4_VEHICLE_COMMAND.VEHICLE_CMD_RESULT_UNSUPPORTED)
    | %         tune_negative(true);
    |         
    |     otherwise
    | end
    | 
    | % publish ACK
    | command_ack_out_.command = cmd_in.command;
    | command_ack_out_.result = result;
    | command_ack_out_.target_system = cmd_in.source_system;
    | command_ack_out_.target_component = cmd_in.source_component;
    | command_ack_out_.timestamp = uint64(getSimulationTime * 1e+6);
    | 
    | end
  function evaluate_prearm_status:
    | function evaluate_prearm_status()
    | 
    | % if (!_armed.armed && !_status_flags.condition_calibration_enabled) {
    | %     bool preflight_check_res = PreFlightCheck::preflightCheck(nullptr, _status, _status_flags, false, true,
    | %     hrt_elapsed_time(&_boot_timestamp));
    | %     
    | %     // skip arm authorization check until actual arming attempt
    | %     PreFlightCheck::arm_requirements_t arm_req = _arm_requirements;
    | %     arm_req.arm_authorization = false;
    | %     bool prearm_check_res = PreFlightCheck::preArmCheck(nullptr, _status_flags, _safety, arm_req, _status, false);
    | %     
    | %     set_health_flags(subsystem_info_s::SUBSYSTEM_TYPE_PREARM_CHECK, true, true, (preflight_check_res
    | %     && prearm_check_res), _status);
    | %     }
    | 
    | end
  function ret = stabilization_required:
    | function ret = stabilization_required()
    | 
    | ret = (vehicle_status_out_.vehicle_type == PX4_VEHICLE_STATUS.VEHICLE_TYPE_ROTARY_WING || ...   % is a rotary wing, or
    |     vehicle_status_out_.vtol_fw_permanent_stab || ...                                           % is a VTOL in fixed wing mode and stabilisation is on, or
    |     (vtol_status.vtol_in_trans_mode && ...                                                      % is currently a VTOL transitioning AND
    |     vehicle_status_out_.vehicle_type == PX4_VEHICLE_STATUS.VEHICLE_TYPE_FIXED_WING));           % is a fixed wing, ie: transitioning back to rotary wing mode
    | 
    | end
  function set_offboard_flags:
    | function set_offboard_flags()
    | 
    | control_mode_out_.flag_control_offboard_enabled = true;
    | 
    | if offboard_control_mode.position
    |     control_mode_out_.flag_control_position_enabled = true;
    |     control_mode_out_.flag_control_velocity_enabled = true;
    |     control_mode_out_.flag_control_altitude_enabled = true;
    |     control_mode_out_.flag_control_climb_rate_enabled = true;
    |     control_mode_out_.flag_control_acceleration_enabled = true;
    |     control_mode_out_.flag_control_rates_enabled = true;
    |     control_mode_out_.flag_control_attitude_enabled = true;
    | elseif offboard_control_mode.velocity
    |     control_mode_out_.flag_control_velocity_enabled = true;
    |     control_mode_out_.flag_control_altitude_enabled = true;
    |     control_mode_out_.flag_control_climb_rate_enabled = true;
    |     control_mode_out_.flag_control_acceleration_enabled = true;
    |     control_mode_out_.flag_control_rates_enabled = true;
    |     control_mode_out_.flag_control_attitude_enabled = true;
    | elseif offboard_control_mode.acceleration
    |     control_mode_out_.flag_control_acceleration_enabled = true;
    |     control_mode_out_.flag_control_rates_enabled = true;
    |     control_mode_out_.flag_control_attitude_enabled = true;
    | elseif offboard_control_mode.attitude
    |     control_mode_out_.flag_control_rates_enabled = true;
    |     control_mode_out_.flag_control_attitude_enabled = true;
    | elseif offboard_control_mode.body_rate
    |     control_mode_out_.flag_control_rates_enabled = true;
    | end
    | 
    | end
  function ret = main_state_transition(new_main_state):
    | % IMPORTANT: The assumption of callers of this function is that the execution of
    | % this check is essentially "free". Therefore any runtime checking in here has to be
    | % kept super lightweight. No complex logic or calls on external function should be
    | % implemented here.
    | function ret = main_state_transition(new_main_state)
    | 
    | ret = TRANSITION_DENIED;
    | 
    | % transition may be denied even if the same state is requested because conditions may have changed
    | switch (new_main_state)
    |     
    |     case uint8(PX4_COMMANDER_STATE.MAIN_STATE_MAX)
    |         ret = TRANSITION_NOT_CHANGED;
    |         
    |     case {uint8(PX4_COMMANDER_STATE.MAIN_STATE_MANUAL), ...
    |             uint8(PX4_COMMANDER_STATE.MAIN_STATE_STAB), ...
    |             uint8(PX4_COMMANDER_STATE.MAIN_STATE_ACRO)}
    |         ret = TRANSITION_CHANGED;
    |         
    |     case uint8(PX4_COMMANDER_STATE.MAIN_STATE_ALTCTL)
    |         % need at minimum altitude estimate
    |         if vehicle_status_flags_out_.condition_local_altitude_valid || vehicle_status_flags_out_.condition_global_position_valid
    |             ret = TRANSITION_CHANGED;
    |         end
    |         
    |     case uint8(PX4_COMMANDER_STATE.MAIN_STATE_POSCTL)
    |         % need at minimum local position estimate
    |         if vehicle_status_flags_out_.condition_local_position_valid || vehicle_status_flags_out_.condition_global_position_valid
    |             ret = TRANSITION_CHANGED;
    |         end
    |         
    |     case uint8(PX4_COMMANDER_STATE.MAIN_STATE_AUTO_LOITER)
    |         % need global position estimate
    |         if vehicle_status_flags_out_.condition_global_position_valid
    |             ret = TRANSITION_CHANGED;
    |         end
    |         
    |     case {uint8(PX4_COMMANDER_STATE.MAIN_STATE_AUTO_FOLLOW_TARGET), ...
    |             uint8(PX4_COMMANDER_STATE.MAIN_STATE_ORBIT)}
    |         % Follow and orbit only implemented for multicopter
    |         if vehicle_status_out_.vehicle_type == PX4_VEHICLE_STATUS.VEHICLE_TYPE_ROTARY_WING
    |             ret = TRANSITION_CHANGED;
    |         end
    |         
    |     case uint8(PX4_COMMANDER_STATE.MAIN_STATE_AUTO_MISSION)
    |         % need global position, home position, and a valid mission
    |         if vehicle_status_flags_out_.condition_global_position_valid && ...
    |                 vehicle_status_flags_out_.condition_auto_mission_available
    |             ret = TRANSITION_CHANGED;
    |         else
    |             ret = TRANSITION_DENIED;
    |         end
    |         
    |     case uint8(PX4_COMMANDER_STATE.MAIN_STATE_AUTO_RTL)
    |         % need global position and home position
    |         if vehicle_status_flags_out_.condition_global_position_valid && ...
    |                 vehicle_status_flags_out_.condition_home_position_valid
    |             ret = TRANSITION_CHANGED;
    |         end
    |         
    |     case {uint8(PX4_COMMANDER_STATE.MAIN_STATE_AUTO_TAKEOFF), ...
    |             uint8(PX4_COMMANDER_STATE.MAIN_STATE_AUTO_LAND)}
    |         % need local position
    |         if vehicle_status_flags_out_.condition_local_position_valid
    |             ret = TRANSITION_CHANGED;
    |         end
    |         
    |     case uint8(PX4_COMMANDER_STATE.MAIN_STATE_AUTO_PRECLAND)
    |         % need local and global position, and precision land only implemented for multicopters
    |         if vehicle_status_flags_out_.condition_local_position_valid && ...
    |                 vehicle_status_flags_out_.condition_global_position_valid && ...
    |                 vehicle_status_out_.vehicle_type == PX4_VEHICLE_STATUS.VEHICLE_TYPE_ROTARY_WING
    |             ret = TRANSITION_CHANGED;
    |         end
    |         
    |     case uint8(PX4_COMMANDER_STATE.MAIN_STATE_OFFBOARD)
    |         % need offboard signal
    |         if ~vehicle_status_flags_out_.offboard_control_signal_lost
    |             ret = TRANSITION_CHANGED;
    |         end
    |         
    | end
    | 
    | %% result
    | if ret == TRANSITION_CHANGED
    |     if internal_state_out_.main_state ~= uint8(new_main_state)
    |         internal_state_out_.main_state = uint8(new_main_state);
    |         internal_state_out_.main_state_changes = internal_state_out_.main_state_changes + 1;
    |         internal_state_out_.timestamp = uint64(getSimulationTime * 1e+6);
    |     else
    |         ret = TRANSITION_NOT_CHANGED;
    |     end
    | end
    | 
    | end
